simulink model "blast_module_casperize"  (R2019a)
settings: Solver=VariableStepDiscrete  StartTime=0.0  StopTime=10.0  RelTol=1e-3
undefined symbols (not defined in the file): I, pfb_coeff_gen_calc, Q
libraries: xbsIndex_r4 x5938, casper_library_misc x46, casper_library_delays x20, xrbsSSR_Library x9, xps_library x2, casper_library_reorder x2
(part 1 of 83)
settings Model: Creator=root  LastModifiedBy=jackh
settings DataIOCC: LimitDataPoints=on  SaveFormat=Array  ReturnWorkspaceOutputs=off
settings OptimizationCC: DefaultParameterBehavior=Inlined  ExpressionDepthLimit=2147483647  LifeSpan=inf
settings DebuggingCC: UnderspecifiedInitializationDetection=Classic  MergeDetectMultiDrivingBlocksExec=none  SolverPrmCheckMsg=warning  StateNameClashWarn=warning  PregeneratedLibrarySubsystemCodeDiagnostic=none  SFUnexpectedBacktrackingDiag=warning  SFNoUnconditionalDefaultTransitionDiag=warning  SFExecutionAtInitializationDiag=none  ArithmeticOperatorsInVariantConditions=warning
settings HardwareCC: ProdBitPerPointer=32  ProdBitPerSizeT=32  ProdBitPerPtrDiffT=32  ProdLargestAtomicFloat=None  ProdIntDivRoundTo=Undefined  ProdEndianess=Unspecified  ProdWordSize=32  ProdHWDeviceType=32-bit Generic
settings ModelReferenceCC: PropagateSignalLabelsOutOfModel=off
settings SFSimCC: SimUseLocalCustomCode=off
settings RTWCC: RTWUseLocalCustomCode=off
settings CodeAppCC: StateflowObjectComments=on
settings GRTTargetCC: TargetLangStandard=C89/C90 (ANSI)  GeneratePreprocessorConditionals=Disable all
settings ConfigComp: CovMetricSettings=dw  CovHtmlReporting=on  CovSaveCumulativeToWorkspaceVar=on  CovSaveSingleToWorkspaceVar=on  CovExternalEMLEnable=off

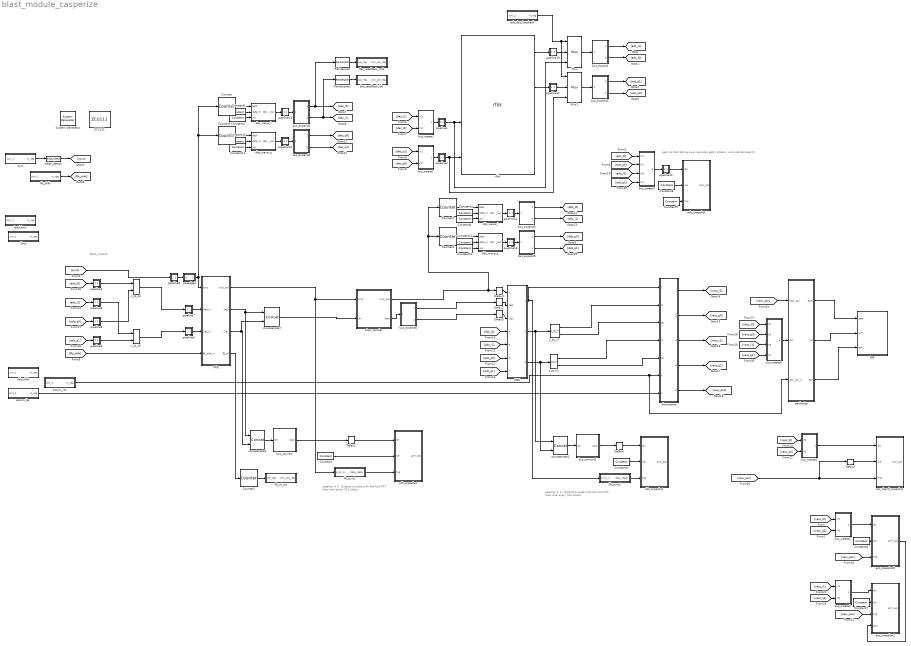
== system blast_module_casperize ==
  note: pack so that taking even samples gets I stream, and odd samples Q
  note: blast_module
  note: Latency = 2. Outputs a pulse with the first FFT,
      | then one every 512 clocks
  note: Latency = 2. Outputs a pulse with the first FFT,
      | then one every 512 clocks
  " System Generator" : xbsIndex_r4/ System Generator  Tag=genX  xilinxfamily=zynquplusRFSOC  part=xczu28dr  speed=-2-e  package=ffvg1517  synthesis_tool=XST  clock_wrapper=Clock Enables  directory=/home/jackh/src/umanc/souk/blast_module_casperize/sysgen  proj_type=Vivado  Synth_file=Vivado Synthesis Defaults  Impl_file=Vivado Implementation Defaults  testbench=off  simulink_period=1  sysclk_period=4.069  dcm_input_clock_period=10  incr_netlist=off  trim_vbits=Everywhere in SubSystem  dbl_ovrd=According to Block Masks  core_generation=According to Block Masks  run_coregen=off  deprecated_control=off  eval_field=0  block_type=sysgen
  Constant{,5..9} (6 alike) : xbsIndex_r4/Constant  const=1.0  gui_display_data_type=Boolean  arith_type=Boolean  n_bits=16  bin_pt=14  preci_type=Single  exp_width=8  frac_width=24  explicit_period=on  period=1  equ=P=C  opselect=C  inp2=PCIN>>17  opr=+  inp1=P  carry=CIN  dbl_ovrd=off  block_type=constant
  Constant{1,3,10,12} (4 alike) : xbsIndex_r4/Constant  const=0  gui_display_data_type=Fixed-point  arith_type=Unsigned  n_bits=32  bin_pt=0  preci_type=Single  exp_width=8  frac_width=24  explicit_period=on  period=1  equ=P=C  opselect=C  inp2=PCIN>>17  opr=+  inp1=P  carry=CIN  dbl_ovrd=off  block_type=constant
  Constant{2,4,11,13} (4 alike) : xbsIndex_r4/Constant  const=0  gui_display_data_type=Boolean  arith_type=Boolean  n_bits=64  bin_pt=0  preci_type=Single  exp_width=8  frac_width=24  explicit_period=on  period=1  equ=P=C  opselect=C  inp2=PCIN>>17  opr=+  inp1=P  carry=CIN  dbl_ovrd=off  block_type=constant
  Counter{,1,3..4} (4 alike) : xbsIndex_r4/Counter  cnt_type=Free Running  cnt_to=Inf  operation=Up  start_count=0  cnt_by_val=1  arith_type=Unsigned  n_bits=17  bin_pt=0  load_pin=off  rst=on  en=off  explicit_period=on  period=1  use_behavioral_HDL=off  implementation=Fabric  dbl_ovrd=off  block_type=counter
  Counter2 : xbsIndex_r4/Counter  cnt_type=Free Running  cnt_to=Inf  operation=Up  start_count=0  cnt_by_val=1  arith_type=Unsigned  n_bits=32  bin_pt=0  load_pin=off  rst=off  en=on  explicit_period=on  period=1  use_behavioral_HDL=off  implementation=Fabric  dbl_ovrd=off  block_type=counter
  DDC : Subsystem
  Delay{1..5} (5 alike) : xbsIndex_r4/Delay  rst=off  infoeditControl=Selection of Reset will increase slice count due to use of real FFs and instead of SRLs  en=off  latency=2  reg_retiming=off  dbl_ovrd=off  block_type=delay
      settings: SourceProductName=Attempt to write the readonly database /home/ugrad/.matlab/R2018a/slblocks_master.db. (attempt to write a readonly database)  xl_area=[18 36 0 0 0 0 0]
  Delay9 : xbsIndex_r4/Delay  rst=off  infoeditControl=Selection of Reset will increase slice count due to use of real FFs and instead of SRLs  en=off  latency=1  reg_retiming=off  dbl_ovrd=off  block_type=delay
      settings: SourceProductName=Attempt to write the readonly database /home/ugrad/.matlab/R2018a/slblocks_master.db. (attempt to write a readonly database)  xl_area=[18 36 0 0 0 0 0]
  Mux : xbsIndex_r4/Mux  inputs=2  en=off  latency=1  precision=Full  arith_type=Unsigned  n_bits=16  bin_pt=14  quantization=Truncate  overflow=Wrap  dbl_ovrd=off  block_type=mux
  Mux1 : xbsIndex_r4/Mux  inputs=2  en=off  latency=1  precision=Full  arith_type=Unsigned  n_bits=16  bin_pt=14  quantization=Truncate  overflow=Wrap  dbl_ovrd=off  block_type=mux
  PFB : Subsystem
  Reinterpret : xbsIndex_r4/Reinterpret  force_arith_type=on  arith_type=Unsigned  force_bin_pt=on  bin_pt=0  block_type=reinterpret
  Reinterpret1 : xbsIndex_r4/Reinterpret  force_arith_type=on  arith_type=Unsigned  force_bin_pt=on  bin_pt=0  block_type=reinterpret
  ZCU111 : xps_library/Platforms/ZCU111  Tag=xps:xsg  hw_sys=ZCU111:xczu28dr  clk_src=adc_clk  clk_rate=245.76  pl_clk_rate=122.88  sample_period=1  synthesis_tool=XST
      settings: SourceProductName=CASPER XPS Blockset
  acc_chan0_snapshot : Subsystem  Tag=casper:snapshot  AncestorBlock=casper_library_scopes/snapshot  mask(snapshot){storage=bram, dram_dimm=2, dram_clock=250, nsamples=13, data_width=64, offset=off, circap=off, value=off, ext_arm=off, ext_circ=off, provide_outputs=on, use_dsp48=off}
      mask prompts: storage "Storage medium"; dram_dimm "DRAM dimm"; dram_clock "DRAM clock rate"; nsamples "Number of Samples (2^?)"; data_width "Data width"; offset "Start delay support"; circap "Circular capture support"; value "Extra value capture support"; ext_arm "External arm support"; ext_circ "External circular capture support"; provide_outputs "Provide outputs"; use_dsp48 "Use DSP48s to implement counters"
      mask help:
      | Standard snap block, but with the following optional extras;
      |  1) Optionally delay the fabric trigger by a user-specified number of valids.
      |  2) Capture continuously after a trigger until a stop pulse is received. Data is captured into BRAM continuously, with old data being overwritten until a stop command is received. Then stop capturing when memory is filled. This enables you to get some data before and some data after the stop pulse. Use the 'tr_en_cnt' register to determine where you are in your vector. 'Addr' register's MSb now indicates 'busy capturing'.
      |  3) Optionally capture a value on an input port to a register at the same time as the first data sample.
      |  4) Implement counters using DSP48Es to save resources.
      mask init:
      | snapshot_init(gcb, ...
      |     'storage', storage, ...
      |     'dram_dimm', dram_dimm, ...
      |     'dram_clock', dram_clock, ...
      |     'nsamples', nsamples, ...
      |     'data_width', data_width, ...
      |     'offset', offset, ...
      |     'circap', circap, ...
      |     'value', value, ...
      |     'ext_arm', ext_arm, ...
      |     'ext_circ', ext_circ, ...
      |     'provide_outputs', 'off', ...
      |     'use_dsp48', use_dsp48);
      settings: AttributesFormatString=|
      | 64 wide, 8192 deep
      | debugID: 9255584
      mask TypeOptions storage: bram | dram
      mask Callback storage: snapshot_callback();
      mask TypeOptions dram_dimm: 1 | 2 | 3 | 4
      mask TypeOptions dram_clock: 200 | 250 | 266 | 300 | 333
      mask TypeOptions data_width: 8 | 16 | 32 | 64 | 128
  acc_snapshot0 : Subsystem  Tag=casper:snapshot  AncestorBlock=casper_library_scopes/snapshot  mask(snapshot){storage=bram, dram_dimm=2, dram_clock=250, nsamples=10, data_width=64, offset=off, circap=off, value=off, ext_arm=off, ext_circ=off, provide_outputs=on, use_dsp48=off}
      mask prompts: storage "Storage medium"; dram_dimm "DRAM dimm"; dram_clock "DRAM clock rate"; nsamples "Number of Samples (2^?)"; data_width "Data width"; offset "Start delay support"; circap "Circular capture support"; value "Extra value capture support"; ext_arm "External arm support"; ext_circ "External circular capture support"; provide_outputs "Provide outputs"; use_dsp48 "Use DSP48s to implement counters"
      mask help:
      | Standard snap block, but with the following optional extras;
      |  1) Optionally delay the fabric trigger by a user-specified number of valids.
      |  2) Capture continuously after a trigger until a stop pulse is received. Data is captured into BRAM continuously, with old data being overwritten until a stop command is received. Then stop capturing when memory is filled. This enables you to get some data before and some data after the stop pulse. Use the 'tr_en_cnt' register to determine where you are in your vector. 'Addr' register's MSb now indicates 'busy capturing'.
      |  3) Optionally capture a value on an input port to a register at the same time as the first data sample.
      |  4) Implement counters using DSP48Es to save resources.
      mask init: same as blast_module_casperize/acc_chan0_snapshot
      settings: AttributesFormatString=|
      | 64 wide, 1024 deep
      | debugID: 50070968
      mask TypeOptions storage: bram | dram
      mask Callback storage: snapshot_callback();
      mask TypeOptions dram_dimm: 1 | 2 | 3 | 4
      mask TypeOptions dram_clock: 200 | 250 | 266 | 300 | 333
      mask TypeOptions data_width: 8 | 16 | 32 | 64 | 128
  acc_snapshot1 : Subsystem  Tag=casper:snapshot  AncestorBlock=casper_library_scopes/snapshot  mask(snapshot){storage=bram, dram_dimm=2, dram_clock=250, nsamples=10, data_width=64, offset=off, circap=off, value=off, ext_arm=on, ext_circ=off, provide_outputs=on, use_dsp48=off}
      mask prompts: storage "Storage medium"; dram_dimm "DRAM dimm"; dram_clock "DRAM clock rate"; nsamples "Number of Samples (2^?)"; data_width "Data width"; offset "Start delay support"; circap "Circular capture support"; value "Extra value capture support"; ext_arm "External arm support"; ext_circ "External circular capture support"; provide_outputs "Provide outputs"; use_dsp48 "Use DSP48s to implement counters"
      mask help:
      | Standard snap block, but with the following optional extras;
      |  1) Optionally delay the fabric trigger by a user-specified number of valids.
      |  2) Capture continuously after a trigger until a stop pulse is received. Data is captured into BRAM continuously, with old data being overwritten until a stop command is received. Then stop capturing when memory is filled. This enables you to get some data before and some data after the stop pulse. Use the 'tr_en_cnt' register to determine where you are in your vector. 'Addr' register's MSb now indicates 'busy capturing'.
      |  3) Optionally capture a value on an input port to a register at the same time as the first data sample.
      |  4) Implement counters using DSP48Es to save resources.
      mask init: same as blast_module_casperize/acc_chan0_snapshot
      settings: AttributesFormatString=|
      | 64 wide, 1024 deep
      | debugID: 50070969
      mask TypeOptions storage: bram | dram
      mask Callback storage: snapshot_callback();
      mask TypeOptions dram_dimm: 1 | 2 | 3 | 4
      mask TypeOptions dram_clock: 200 | 250 | 266 | 300 | 333
      mask TypeOptions data_width: 8 | 16 | 32 | 64 | 128
  accum_len : Subsystem  Tag=xps:sw_reg  AncestorBlock=xps_library/Memory/software_register  mask(swreg){io_dir=From Processor, io_delay=0, init_val=0, sample_period=1, names=reg, bitwidths=24, bin_pts=0, arith_types=0, sim_port=on, show_format=on}
      mask prompts: io_dir "I/O direction"; io_delay "I/O delay"; init_val "Initial Value"; sample_period "Sample period"; names "Bitfield names [msb...lsb]"; bitwidths "Bitfield widths"; bin_pts "Bitfield binary pts"; arith_types "Bitfield types, ufix=0, fix=1, bool=2"; sim_port "Provide sim input/output?"; show_format "Print format string?"
      mask help: A 32-bit software-accessible register. Can be divided into bitfields of varying widths and types using the fields in the block mask.
      mask init:
      | swreg_init(gcb)
      settings: AttributesFormatString=1input:uf24.0 = 24 bits
      mask TypeOptions io_dir: To Processor | From Processor
      mask Callback io_dir:
      | mask_enables = get_param(gcb, 'MaskEnables');
      | mask_names = get_param(gcb, 'MaskNames');
      | if strcmp(get_param(gcb, 'io_dir'), 'To Processor'),
      |     mask_enables{ismember(mask_names, 'sample_period')} = 'off';
      | else
      |     mask_enables{ismember(mask_names, 'sample_period')} = 'on';
      | end
      | set_param(gcb, 'MaskEnables', mask_enables);
      mask DialogControl ParameterTabVar0 Prompt: Setup
  accum_rst : Subsystem  Tag=xps:sw_reg  AncestorBlock=xps_library/Memory/software_register  mask(swreg){io_dir=From Processor, io_delay=0, init_val=0, sample_period=1, names=reg, bitwidths=1, bin_pts=0, arith_types=2, sim_port=on, show_format=on}
      mask prompts: io_dir "I/O direction"; io_delay "I/O delay"; init_val "Initial Value"; sample_period "Sample period"; names "Bitfield names [msb...lsb]"; bitwidths "Bitfield widths"; bin_pts "Bitfield binary pts"; arith_types "Bitfield types, ufix=0, fix=1, bool=2"; sim_port "Provide sim input/output?"; show_format "Print format string?"
      mask help: A 32-bit software-accessible register. Can be divided into bitfields of varying widths and types using the fields in the block mask.
      mask init:
      | swreg_init(gcb)
      settings: AttributesFormatString=1input:b = 1 bits
      mask TypeOptions io_dir: To Processor | From Processor
      mask Callback io_dir:
      | mask_enables = get_param(gcb, 'MaskEnables');
      | mask_names = get_param(gcb, 'MaskNames');
      | if strcmp(get_param(gcb, 'io_dir'), 'To Processor'),
      |     mask_enables{ismember(mask_names, 'sample_period')} = 'off';
      | else
      |     mask_enables{ismember(mask_names, 'sample_period')} = 'on';
      | end
      | set_param(gcb, 'MaskEnables', mask_enables);
      mask DialogControl ParameterTabVar0 Prompt: Setup
  adc_dac_loopback : Subsystem  Tag=xps:sw_reg  AncestorBlock=xps_library/Memory/software_register  mask(swreg){io_dir=From Processor, io_delay=0, init_val=0, sample_period=1, names=reg, bitwidths=1, bin_pts=0, arith_types=0, sim_port=on, show_format=on}
      mask prompts: io_dir "I/O direction"; io_delay "I/O delay"; init_val "Initial Value"; sample_period "Sample period"; names "Bitfield names [msb...lsb]"; bitwidths "Bitfield widths"; bin_pts "Bitfield binary pts"; arith_types "Bitfield types, ufix=0, fix=1, bool=2"; sim_port "Provide sim input/output?"; show_format "Print format string?"
      mask help: A 32-bit software-accessible register. Can be divided into bitfields of varying widths and types using the fields in the block mask.
      mask init:
      | swreg_init(gcb)
      settings: AttributesFormatString=1input:uf1.0 = 1 bits
      mask TypeOptions io_dir: To Processor | From Processor
      mask Callback io_dir:
      | mask_enables = get_param(gcb, 'MaskEnables');
      | mask_names = get_param(gcb, 'MaskNames');
      | if strcmp(get_param(gcb, 'io_dir'), 'To Processor'),
      |     mask_enables{ismember(mask_names, 'sample_period')} = 'off';
      | else
      |     mask_enables{ismember(mask_names, 'sample_period')} = 'on';
      | end
      | set_param(gcb, 'MaskEnables', mask_enables);
      mask DialogControl ParameterTabVar0 Prompt: Setup
  adc_snapshot : Subsystem  Tag=casper:snapshot  AncestorBlock=casper_library_scopes/snapshot  mask(snapshot){storage=bram, dram_dimm=2, dram_clock=250, nsamples=11, data_width=64, offset=off, circap=off, value=off, ext_arm=off, ext_circ=off, provide_outputs=on, use_dsp48=off}
      mask prompts: storage "Storage medium"; dram_dimm "DRAM dimm"; dram_clock "DRAM clock rate"; nsamples "Number of Samples (2^?)"; data_width "Data width"; offset "Start delay support"; circap "Circular capture support"; value "Extra value capture support"; ext_arm "External arm support"; ext_circ "External circular capture support"; provide_outputs "Provide outputs"; use_dsp48 "Use DSP48s to implement counters"
      mask help:
      | Standard snap block, but with the following optional extras;
      |  1) Optionally delay the fabric trigger by a user-specified number of valids.
      |  2) Capture continuously after a trigger until a stop pulse is received. Data is captured into BRAM continuously, with old data being overwritten until a stop command is received. Then stop capturing when memory is filled. This enables you to get some data before and some data after the stop pulse. Use the 'tr_en_cnt' register to determine where you are in your vector. 'Addr' register's MSb now indicates 'busy capturing'.
      |  3) Optionally capture a value on an input port to a register at the same time as the first data sample.
      |  4) Implement counters using DSP48Es to save resources.
      mask init: same as blast_module_casperize/acc_chan0_snapshot
      settings: AttributesFormatString=|
      | 64 wide, 2048 deep
      | debugID: 118348857
      mask TypeOptions storage: bram | dram
      mask Callback storage: snapshot_callback();
      mask TypeOptions dram_dimm: 1 | 2 | 3 | 4
      mask TypeOptions dram_clock: 200 | 250 | 266 | 300 | 333
      mask TypeOptions data_width: 8 | 16 | 32 | 64 | 128
  bins : Subsystem  Tag=xps:sw_reg  AncestorBlock=xps_library/Memory/software_register  mask(swreg){io_dir=From Processor, io_delay=0, init_val=0, sample_period=1, names=reg, bitwidths=10, bin_pts=0, arith_types=0, sim_port=on, show_format=on}
      mask prompts: io_dir "I/O direction"; io_delay "I/O delay"; init_val "Initial Value"; sample_period "Sample period"; names "Bitfield names [msb...lsb]"; bitwidths "Bitfield widths"; bin_pts "Bitfield binary pts"; arith_types "Bitfield types, ufix=0, fix=1, bool=2"; sim_port "Provide sim input/output?"; show_format "Print format string?"
      mask help: A 32-bit software-accessible register. Can be divided into bitfields of varying widths and types using the fields in the block mask.
      mask init:
      | swreg_init(gcb)
      settings: AttributesFormatString=1input:uf10.0 = 10 bits
      mask TypeOptions io_dir: To Processor | From Processor
      mask Callback io_dir:
      | mask_enables = get_param(gcb, 'MaskEnables');
      | mask_names = get_param(gcb, 'MaskNames');
      | if strcmp(get_param(gcb, 'io_dir'), 'To Processor'),
      |     mask_enables{ismember(mask_names, 'sample_period')} = 'off';
      | else
      |     mask_enables{ismember(mask_names, 'sample_period')} = 'on';
      | end
      | set_param(gcb, 'MaskEnables', mask_enables);
      mask DialogControl ParameterTabVar0 Prompt: Setup
  bus_convert : Subsystem  AncestorBlock=casper_library_bus/bus_convert  mask(bus_convert){n_bits_in=[18 18 18 18], bin_pt_in=[17 17 17 17], cmplx=off, n_bits_out=16, bin_pt_out=15, quantization=0, overflow=0, csp_latency=0, of=off, misc=off}
      mask prompts: n_bits_in "input bit widths"; bin_pt_in "input binary points"; cmplx "input complex"; n_bits_out "output bit widths"; bin_pt_out "output binary points"; quantization "quantization strategy (Truncate=0, Round  (unbiased: +/- Inf)=1, Round (unbiased: Even Values)=2)"; overflow "overflow strategy (Wrap=0, Saturate=1, Flag as error=2)"; csp_latency "latency"; of "overflow indication"; misc "misc support"
      mask help: Convert components of busses
      mask init:
      | bus_convert_init(gcb, ...
      |     'n_bits_in', n_bits_in, ...
      |     'bin_pt_in', bin_pt_in, ...
      |     'cmplx', cmplx, ...
      |     'n_bits_out', n_bits_out, ...
      |     'bin_pt_out', bin_pt_out, ...
      |     'quantization', quantization, ...
      |     'overflow', overflow, ...
      |     'csp_latency', csp_latency, ...
      |     'misc', misc, ...
      |     'of', of);
  bus_convert1 : Subsystem  AncestorBlock=casper_library_bus/bus_convert  mask(bus_convert){n_bits_in=[19 19 19 19], bin_pt_in=[18 18 18 18], cmplx=off, n_bits_out=16, bin_pt_out=15, quantization=0, overflow=0, csp_latency=0, of=off, misc=off}
      mask prompts: n_bits_in "input bit widths"; bin_pt_in "input binary points"; cmplx "input complex"; n_bits_out "output bit widths"; bin_pt_out "output binary points"; quantization "quantization strategy (Truncate=0, Round  (unbiased: +/- Inf)=1, Round (unbiased: Even Values)=2)"; overflow "overflow strategy (Wrap=0, Saturate=1, Flag as error=2)"; csp_latency "latency"; of "overflow indication"; misc "misc support"
      mask help: Convert components of busses
      mask init: same as blast_module_casperize/bus_convert
  bus_create : Subsystem  AncestorBlock=casper_library_flow_control/bus_create  mask(bus_create){inputNum=2}
      mask prompts: inputNum "Number of inputs:"
      mask init:
      | bus_create_init(gcb,...
      |     'inputNum', inputNum);
  bus_create1 : Subsystem  AncestorBlock=casper_library_flow_control/bus_create  mask(bus_create){inputNum=2}
      mask prompts: inputNum "Number of inputs:"
      mask init:
      | bus_create_init(gcb,...
      |     'inputNum', inputNum);
  bus_create2 : Subsystem  AncestorBlock=casper_library_flow_control/bus_create  mask(bus_create){inputNum=2}
      mask prompts: inputNum "Number of inputs:"
      mask init:
      | bus_create_init(gcb,...
      |     'inputNum', inputNum);
  bus_create3 : Subsystem  AncestorBlock=casper_library_flow_control/bus_create  mask(bus_create){inputNum=2}
      mask prompts: inputNum "Number of inputs:"
      mask init:
      | bus_create_init(gcb,...
      |     'inputNum', inputNum);
  bus_create4 : Subsystem  AncestorBlock=casper_library_flow_control/bus_create  mask(bus_create){inputNum=4}
      mask prompts: inputNum "Number of inputs:"
      mask init:
      | bus_create_init(gcb,...
      |     'inputNum', inputNum);
  bus_create5 : Subsystem  AncestorBlock=casper_library_flow_control/bus_create  mask(bus_create){inputNum=2}
      mask prompts: inputNum "Number of inputs:"
      mask init:
      | bus_create_init(gcb,...
      |     'inputNum', inputNum);
  bus_create6 : Subsystem  AncestorBlock=casper_library_flow_control/bus_create  mask(bus_create){inputNum=4}
      mask prompts: inputNum "Number of inputs:"
      mask init:
      | bus_create_init(gcb,...
      |     'inputNum', inputNum);
  bus_expand : Subsystem  AncestorBlock=casper_library_flow_control/bus_expand  mask(bus_expand){mode=divisions of equal size, outputNum=2, outputWidth=16, outputBinaryPt=15, outputArithmeticType=1, show_format=off, outputToWorkspace=off, variablePrefix=out, outputToModelAsWell=on}
      mask prompts: outputNum "Number of outputs:"; outputWidth "Output width:"; outputBinaryPt "Output binary point position:"; outputArithmeticType "Output arithmetic type (ufix=0, fix=1, bool=2):"; show_format "Print format string?"; outputToWorkspace "Output to workspace?"; variablePrefix "Variable name prefix:"; outputToModelAsWell "Output to model as well?"
      mask help:
      | Expands a 'bus' made using a bus_create or Xilinx
      | concat block.
      | The input will be divided into the specified number
      | of outputs with the specified arithmetic types.
      | Divisions are made from most significant bit.
      mask init:
      | bus_expand_init(gcb,...
      |     'mode', mode, ...
      |     'outputNum', outputNum, ...
      |     'outputWidth', outputWidth, ...
      |     'outputBinaryPt', outputBinaryPt, ...
      |     'outputArithmeticType', outputArithmeticType, ...
      |     'show_format', show_format, ...
      |     'outputToWorkspace', outputToWorkspace, ...
      |     'variablePrefix', variablePrefix, ...
      |     'outputToModelAsWell', outputToModelAsWell);
      settings: AttributesFormatString=2 outputs
      mask TypeOptions mode: divisions of equal size | divisions of arbitrary size
      mask Callback mode: bus_expand_callback();
      mask Callback outputWidth: bus_expand_callback();
      mask Callback outputToWorkspace: bus_expand_callback();
  bus_expand1 : Subsystem  AncestorBlock=casper_library_flow_control/bus_expand  mask(bus_expand){mode=divisions of equal size, outputNum=2, outputWidth=16, outputBinaryPt=15, outputArithmeticType=1, show_format=off, outputToWorkspace=off, variablePrefix=out, outputToModelAsWell=on}
      mask prompts: outputNum "Number of outputs:"; outputWidth "Output width:"; outputBinaryPt "Output binary point position:"; outputArithmeticType "Output arithmetic type (ufix=0, fix=1, bool=2):"; show_format "Print format string?"; outputToWorkspace "Output to workspace?"; variablePrefix "Variable name prefix:"; outputToModelAsWell "Output to model as well?"
      mask help:
      | Expands a 'bus' made using a bus_create or Xilinx
      | concat block.
      | The input will be divided into the specified number
      | of outputs with the specified arithmetic types.
      | Divisions are made from most significant bit.
      mask init: same as blast_module_casperize/bus_expand
      settings: AttributesFormatString=2 outputs
      mask TypeOptions mode: divisions of equal size | divisions of arbitrary size
      mask Callback mode: bus_expand_callback();
      mask Callback outputWidth: bus_expand_callback();
      mask Callback outputToWorkspace: bus_expand_callback();
  bus_expand2 : Subsystem  AncestorBlock=casper_library_flow_control/bus_expand  mask(bus_expand){mode=divisions of equal size, outputNum=2, outputWidth=16, outputBinaryPt=15, outputArithmeticType=1, show_format=off, outputToWorkspace=off, variablePrefix=out, outputToModelAsWell=on}
      mask prompts: outputNum "Number of outputs:"; outputWidth "Output width:"; outputBinaryPt "Output binary point position:"; outputArithmeticType "Output arithmetic type (ufix=0, fix=1, bool=2):"; show_format "Print format string?"; outputToWorkspace "Output to workspace?"; variablePrefix "Variable name prefix:"; outputToModelAsWell "Output to model as well?"
      mask help:
      | Expands a 'bus' made using a bus_create or Xilinx
      | concat block.
      | The input will be divided into the specified number
      | of outputs with the specified arithmetic types.
      | Divisions are made from most significant bit.
      mask init: same as blast_module_casperize/bus_expand
      settings: AttributesFormatString=2 outputs
      mask TypeOptions mode: divisions of equal size | divisions of arbitrary size
      mask Callback mode: bus_expand_callback();
      mask Callback outputWidth: bus_expand_callback();
      mask Callback outputToWorkspace: bus_expand_callback();
  bus_expand3 : Subsystem  AncestorBlock=casper_library_flow_control/bus_expand  mask(bus_expand){mode=divisions of equal size, outputNum=2, outputWidth=16, outputBinaryPt=15, outputArithmeticType=1, show_format=off, outputToWorkspace=off, variablePrefix=out, outputToModelAsWell=on}
      mask prompts: outputNum "Number of outputs:"; outputWidth "Output width:"; outputBinaryPt "Output binary point position:"; outputArithmeticType "Output arithmetic type (ufix=0, fix=1, bool=2):"; show_format "Print format string?"; outputToWorkspace "Output to workspace?"; variablePrefix "Variable name prefix:"; outputToModelAsWell "Output to model as well?"
      mask help:
      | Expands a 'bus' made using a bus_create or Xilinx
      | concat block.
      | The input will be divided into the specified number
      | of outputs with the specified arithmetic types.
      | Divisions are made from most significant bit.
      mask init: same as blast_module_casperize/bus_expand
      settings: AttributesFormatString=2 outputs
      mask TypeOptions mode: divisions of equal size | divisions of arbitrary size
      mask Callback mode: bus_expand_callback();
      mask Callback outputWidth: bus_expand_callback();
      mask Callback outputToWorkspace: bus_expand_callback();
  bus_expand4 : Subsystem  AncestorBlock=casper_library_flow_control/bus_expand  mask(bus_expand){mode=divisions of equal size, outputNum=2, outputWidth=16, outputBinaryPt=15, outputArithmeticType=1, show_format=off, outputToWorkspace=off, variablePrefix=out, outputToModelAsWell=on}
      mask prompts: outputNum "Number of outputs:"; outputWidth "Output width:"; outputBinaryPt "Output binary point position:"; outputArithmeticType "Output arithmetic type (ufix=0, fix=1, bool=2):"; show_format "Print format string?"; outputToWorkspace "Output to workspace?"; variablePrefix "Variable name prefix:"; outputToModelAsWell "Output to model as well?"
      mask help:
      | Expands a 'bus' made using a bus_create or Xilinx
      | concat block.
      | The input will be divided into the specified number
      | of outputs with the specified arithmetic types.
      | Divisions are made from most significant bit.
      mask init: same as blast_module_casperize/bus_expand
      settings: AttributesFormatString=2 outputs
      mask TypeOptions mode: divisions of equal size | divisions of arbitrary size
      mask Callback mode: bus_expand_callback();
      mask Callback outputWidth: bus_expand_callback();
      mask Callback outputToWorkspace: bus_expand_callback();
  bus_expand5 : Subsystem  AncestorBlock=casper_library_flow_control/bus_expand  mask(bus_expand){mode=divisions of equal size, outputNum=2, outputWidth=16, outputBinaryPt=15, outputArithmeticType=1, show_format=off, outputToWorkspace=off, variablePrefix=out, outputToModelAsWell=on}
      mask prompts: outputNum "Number of outputs:"; outputWidth "Output width:"; outputBinaryPt "Output binary point position:"; outputArithmeticType "Output arithmetic type (ufix=0, fix=1, bool=2):"; show_format "Print format string?"; outputToWorkspace "Output to workspace?"; variablePrefix "Variable name prefix:"; outputToModelAsWell "Output to model as well?"
      mask help:
      | Expands a 'bus' made using a bus_create or Xilinx
      | concat block.
      | The input will be divided into the specified number
      | of outputs with the specified arithmetic types.
      | Divisions are made from most significant bit.
      mask init: same as blast_module_casperize/bus_expand
      settings: AttributesFormatString=2 outputs
      mask TypeOptions mode: divisions of equal size | divisions of arbitrary size
      mask Callback mode: bus_expand_callback();
      mask Callback outputWidth: bus_expand_callback();
      mask Callback outputToWorkspace: bus_expand_callback();
  bus_expand6 : Subsystem  AncestorBlock=casper_library_flow_control/bus_expand  mask(bus_expand){mode=divisions of equal size, outputNum=2, outputWidth=36, outputBinaryPt=0, outputArithmeticType=0, show_format=off, outputToWorkspace=off, variablePrefix=out, outputToModelAsWell=on}
      mask prompts: outputNum "Number of outputs:"; outputWidth "Output width:"; outputBinaryPt "Output binary point position:"; outputArithmeticType "Output arithmetic type (ufix=0, fix=1, bool=2):"; show_format "Print format string?"; outputToWorkspace "Output to workspace?"; variablePrefix "Variable name prefix:"; outputToModelAsWell "Output to model as well?"
      mask help:
      | Expands a 'bus' made using a bus_create or Xilinx
      | concat block.
      | The input will be divided into the specified number
      | of outputs with the specified arithmetic types.
      | Divisions are made from most significant bit.
      mask init: same as blast_module_casperize/bus_expand
      settings: AttributesFormatString=2 outputs
      mask TypeOptions mode: divisions of equal size | divisions of arbitrary size
      mask Callback mode: bus_expand_callback();
      mask Callback outputWidth: bus_expand_callback();
      mask Callback outputToWorkspace: bus_expand_callback();
  c_to_ri1 : casper_library_misc/c_to_ri  n_bits=19  bin_pt=17
      settings: AttributesFormatString=19_17 r/i  SourceProductName=CASPER DSP Blockset
  c_to_ri7 : casper_library_misc/c_to_ri  n_bits=19  bin_pt=17
      settings: AttributesFormatString=19_17 r/i  SourceProductName=CASPER DSP Blockset
  chan_reorder : Subsystem
  concatenate1 : xbsIndex_r4/Concat  num_inputs=2  dbl_ovrd=off  block_type=concat
      settings: SourceProductName=Attempt to write the readonly database /home/ugrad/.matlab/R2018a/slblocks_master.db. (attempt to write a readonly database)
  concatenate2 : xbsIndex_r4/Concat  num_inputs=2  dbl_ovrd=off  block_type=concat
      settings: SourceProductName=Attempt to write the readonly database /home/ugrad/.matlab/R2018a/slblocks_master.db. (attempt to write a readonly database)
  concatenate7 : xbsIndex_r4/Concat  num_inputs=2  dbl_ovrd=off  block_type=concat
      settings: SourceProductName=Attempt to write the readonly database /home/ugrad/.matlab/R2018a/slblocks_master.db. (attempt to write a readonly database)
  dac_readback_lsb : Subsystem  Tag=xps:sw_reg  AncestorBlock=xps_library/Memory/software_register  mask(swreg){io_dir=To Processor, io_delay=0, init_val=0, sample_period=1, names=reg, bitwidths=16, bin_pts=0, arith_types=0, sim_port=on, show_format=on}
      mask prompts: io_dir "I/O direction"; io_delay "I/O delay"; init_val "Initial Value"; sample_period "Sample period"; names "Bitfield names [msb...lsb]"; bitwidths "Bitfield widths"; bin_pts "Bitfield binary pts"; arith_types "Bitfield types, ufix=0, fix=1, bool=2"; sim_port "Provide sim input/output?"; show_format "Print format string?"
      mask help: A 32-bit software-accessible register. Can be divided into bitfields of varying widths and types using the fields in the block mask.
      mask init:
      | swreg_init(gcb)
      settings: AttributesFormatString=1output:uf16.0 = 16 bits
      mask TypeOptions io_dir: To Processor | From Processor
      mask Callback io_dir:
      | mask_enables = get_param(gcb, 'MaskEnables');
      | mask_names = get_param(gcb, 'MaskNames');
      | if strcmp(get_param(gcb, 'io_dir'), 'To Processor'),
      |     mask_enables{ismember(mask_names, 'sample_period')} = 'off';
      | else
      |     mask_enables{ismember(mask_names, 'sample_period')} = 'on';
      | end
      | set_param(gcb, 'MaskEnables', mask_enables);
      mask DialogControl ParameterTabVar0 Prompt: Setup
  dac_readback_msb : Subsystem  Tag=xps:sw_reg  AncestorBlock=xps_library/Memory/software_register  mask(swreg){io_dir=To Processor, io_delay=0, init_val=0, sample_period=1, names=reg, bitwidths=16, bin_pts=0, arith_types=0, sim_port=on, show_format=on}
      mask prompts: io_dir "I/O direction"; io_delay "I/O delay"; init_val "Initial Value"; sample_period "Sample period"; names "Bitfield names [msb...lsb]"; bitwidths "Bitfield widths"; bin_pts "Bitfield binary pts"; arith_types "Bitfield types, ufix=0, fix=1, bool=2"; sim_port "Provide sim input/output?"; show_format "Print format string?"
      mask help: A 32-bit software-accessible register. Can be divided into bitfields of varying widths and types using the fields in the block mask.
      mask init:
      | swreg_init(gcb)
      settings: AttributesFormatString=1output:uf16.0 = 16 bits
      mask TypeOptions io_dir: To Processor | From Processor
      mask Callback io_dir:
      | mask_enables = get_param(gcb, 'MaskEnables');
      | mask_names = get_param(gcb, 'MaskNames');
      | if strcmp(get_param(gcb, 'io_dir'), 'To Processor'),
      |     mask_enables{ismember(mask_names, 'sample_period')} = 'off';
      | else
      |     mask_enables{ismember(mask_names, 'sample_period')} = 'on';
      | end
      | set_param(gcb, 'MaskEnables', mask_enables);
      mask DialogControl ParameterTabVar0 Prompt: Setup
  dac_wave_i : Subsystem  Tag=xps:bram  AncestorBlock=xps_library/Memory/shared_bram  mask{arith_type=Unsigned, addr_width=17, data_width=32, reg_prim_output=off, reg_core_output=off, optimization=Minimum_Area, data_bin_pt=0, init_vals=[0:2^10-1], sample_rate=1}
      mask prompts: arith_type "Output Data Type"; addr_width "Address width"; data_width "Data Width"; reg_prim_output "Register Primitive Output"; reg_core_output "Register Core Output"; data_bin_pt "Data Binary Point"; init_vals "Initial values (simulation only)"; sample_rate "Sample rate"
      mask init:
      | shared_bram_mask;
      mask TypeOptions arith_type: Unsigned | Signed  (2's comp)
      mask TypeOptions data_width: 8 | 16 | 32 | 64 | 128
      mask TypeOptions optimization: Minimum_Area | Low_Power
  dac_wave_q : Subsystem  Tag=xps:bram  AncestorBlock=xps_library/Memory/shared_bram  mask{arith_type=Unsigned, addr_width=17, data_width=32, reg_prim_output=off, reg_core_output=off, optimization=Minimum_Area, data_bin_pt=0, init_vals=[0:2^10-1], sample_rate=1}
      mask prompts: arith_type "Output Data Type"; addr_width "Address width"; data_width "Data Width"; reg_prim_output "Register Primitive Output"; reg_core_output "Register Core Output"; data_bin_pt "Data Binary Point"; init_vals "Initial values (simulation only)"; sample_rate "Sample rate"
      mask init:
      | shared_bram_mask;
      mask TypeOptions arith_type: Unsigned | Signed  (2's comp)
      mask TypeOptions data_width: 8 | 16 | 32 | 64 | 128
      mask TypeOptions optimization: Minimum_Area | Low_Power
  ddc_snapshot : Subsystem  Tag=casper:snapshot  AncestorBlock=casper_library_scopes/snapshot  mask(snapshot){storage=bram, dram_dimm=2, dram_clock=250, nsamples=12, data_width=64, offset=off, circap=off, value=off, ext_arm=off, ext_circ=off, provide_outputs=on, use_dsp48=off}
      mask prompts: storage "Storage medium"; dram_dimm "DRAM dimm"; dram_clock "DRAM clock rate"; nsamples "Number of Samples (2^?)"; data_width "Data width"; offset "Start delay support"; circap "Circular capture support"; value "Extra value capture support"; ext_arm "External arm support"; ext_circ "External circular capture support"; provide_outputs "Provide outputs"; use_dsp48 "Use DSP48s to implement counters"
      mask help:
      | Standard snap block, but with the following optional extras;
      |  1) Optionally delay the fabric trigger by a user-specified number of valids.
      |  2) Capture continuously after a trigger until a stop pulse is received. Data is captured into BRAM continuously, with old data being overwritten until a stop command is received. Then stop capturing when memory is filled. This enables you to get some data before and some data after the stop pulse. Use the 'tr_en_cnt' register to determine where you are in your vector. 'Addr' register's MSb now indicates 'busy capturing'.
      |  3) Optionally capture a value on an input port to a register at the same time as the first data sample.
      |  4) Implement counters using DSP48Es to save resources.
      mask init: same as blast_module_casperize/acc_chan0_snapshot
      settings: AttributesFormatString=|
      | 64 wide, 4096 deep
      | debugID: 95009402
      mask TypeOptions storage: bram | dram
      mask Callback storage: snapshot_callback();
      mask TypeOptions dram_dimm: 1 | 2 | 3 | 4
      mask TypeOptions dram_clock: 200 | 250 | 266 | 300 | 333
      mask TypeOptions data_width: 8 | 16 | 32 | 64 | 128
  dds_shift : Subsystem  Tag=xps:sw_reg  AncestorBlock=xps_library/Memory/software_register  mask(swreg){io_dir=From Processor, io_delay=0, init_val=0, sample_period=1, names=reg, bitwidths=9, bin_pts=0, arith_types=0, sim_port=on, show_format=on}
      mask prompts: io_dir "I/O direction"; io_delay "I/O delay"; init_val "Initial Value"; sample_period "Sample period"; names "Bitfield names [msb...lsb]"; bitwidths "Bitfield widths"; bin_pts "Bitfield binary pts"; arith_types "Bitfield types, ufix=0, fix=1, bool=2"; sim_port "Provide sim input/output?"; show_format "Print format string?"
      mask help: A 32-bit software-accessible register. Can be divided into bitfields of varying widths and types using the fields in the block mask.
      mask init:
      | swreg_init(gcb)
      settings: AttributesFormatString=1input:uf9.0 = 9 bits
      mask TypeOptions io_dir: To Processor | From Processor
      mask Callback io_dir:
      | mask_enables = get_param(gcb, 'MaskEnables');
      | mask_names = get_param(gcb, 'MaskNames');
      | if strcmp(get_param(gcb, 'io_dir'), 'To Processor'),
      |     mask_enables{ismember(mask_names, 'sample_period')} = 'off';
      | else
      |     mask_enables{ismember(mask_names, 'sample_period')} = 'on';
      | end
      | set_param(gcb, 'MaskEnables', mask_enables);
      mask DialogControl ParameterTabVar0 Prompt: Setup
  dds_wave_i : Subsystem  Tag=xps:bram  AncestorBlock=xps_library/Memory/shared_bram  mask{arith_type=Unsigned, addr_width=17, data_width=32, reg_prim_output=off, reg_core_output=off, optimization=Minimum_Area, data_bin_pt=0, init_vals=[0:2^10-1], sample_rate=1}
      mask prompts: arith_type "Output Data Type"; addr_width "Address width"; data_width "Data Width"; reg_prim_output "Register Primitive Output"; reg_core_output "Register Core Output"; data_bin_pt "Data Binary Point"; init_vals "Initial values (simulation only)"; sample_rate "Sample rate"
      mask init:
      | shared_bram_mask;
      mask TypeOptions arith_type: Unsigned | Signed  (2's comp)
      mask TypeOptions data_width: 8 | 16 | 32 | 64 | 128
      mask TypeOptions optimization: Minimum_Area | Low_Power
  dds_wave_q : Subsystem  Tag=xps:bram  AncestorBlock=xps_library/Memory/shared_bram  mask{arith_type=Unsigned, addr_width=17, data_width=32, reg_prim_output=off, reg_core_output=off, optimization=Minimum_Area, data_bin_pt=0, init_vals=[0:2^10-1], sample_rate=1}
      mask prompts: arith_type "Output Data Type"; addr_width "Address width"; data_width "Data Width"; reg_prim_output "Register Primitive Output"; reg_core_output "Register Core Output"; data_bin_pt "Data Binary Point"; init_vals "Initial values (simulation only)"; sample_rate "Sample rate"
      mask init:
      | shared_bram_mask;
      mask TypeOptions arith_type: Unsigned | Signed  (2's comp)
      mask TypeOptions data_width: 8 | 16 | 32 | 64 | 128
      mask TypeOptions optimization: Minimum_Area | Low_Power
  downsamp : Subsystem
  edge_detect : casper_library_misc/edge_detect  edge=Rising  polarity=Active High  x_in=[0 0.08 0.08 0.16 0.16 0.24 0.24 0.32 0.32 0.4]  y_in="[-1 -1  1  1  1  1  1  1  1  1]"  x_out=[0.6 0.68 0.68 0.76 0.76 0.84 0.84 0.92 0.92 1]  y_out="[-1 -1  1  1 -1 -1 -1 -1 -1 -1]"
  fft_of_cnt : Subsystem  Tag=xps:sw_reg  AncestorBlock=xps_library/Memory/software_register  mask(swreg){io_dir=To Processor, io_delay=0, init_val=0, sample_period=1, names=reg, bitwidths=32, bin_pts=0, arith_types=0, sim_port=on, show_format=on}
      mask prompts: io_dir "I/O direction"; io_delay "I/O delay"; init_val "Initial Value"; sample_period "Sample period"; names "Bitfield names [msb...lsb]"; bitwidths "Bitfield widths"; bin_pts "Bitfield binary pts"; arith_types "Bitfield types, ufix=0, fix=1, bool=2"; sim_port "Provide sim input/output?"; show_format "Print format string?"
      mask help: A 32-bit software-accessible register. Can be divided into bitfields of varying widths and types using the fields in the block mask.
      mask init:
      | swreg_init(gcb)
      settings: AttributesFormatString=1output:uf32.0 = 32 bits
      mask TypeOptions io_dir: To Processor | From Processor
      mask Callback io_dir:
      | mask_enables = get_param(gcb, 'MaskEnables');
      | mask_names = get_param(gcb, 'MaskNames');
      | if strcmp(get_param(gcb, 'io_dir'), 'To Processor'),
      |     mask_enables{ismember(mask_names, 'sample_period')} = 'off';
      | else
      |     mask_enables{ismember(mask_names, 'sample_period')} = 'on';
      | end
      | set_param(gcb, 'MaskEnables', mask_enables);
      mask DialogControl ParameterTabVar0 Prompt: Setup
  fft_shift : Subsystem  Tag=xps:sw_reg  AncestorBlock=xps_library/Memory/software_register  mask(swreg){io_dir=From Processor, io_delay=0, init_val=0, sample_period=1, names=reg, bitwidths=10, bin_pts=0, arith_types=0, sim_port=on, show_format=on}
      mask prompts: io_dir "I/O direction"; io_delay "I/O delay"; init_val "Initial Value"; sample_period "Sample period"; names "Bitfield names [msb...lsb]"; bitwidths "Bitfield widths"; bin_pts "Bitfield binary pts"; arith_types "Bitfield types, ufix=0, fix=1, bool=2"; sim_port "Provide sim input/output?"; show_format "Print format string?"
      mask help: A 32-bit software-accessible register. Can be divided into bitfields of varying widths and types using the fields in the block mask.
      mask init:
      | swreg_init(gcb)
      settings: AttributesFormatString=1input:uf10.0 = 10 bits
      mask TypeOptions io_dir: To Processor | From Processor
      mask Callback io_dir:
      | mask_enables = get_param(gcb, 'MaskEnables');
      | mask_names = get_param(gcb, 'MaskNames');
      | if strcmp(get_param(gcb, 'io_dir'), 'To Processor'),
      |     mask_enables{ismember(mask_names, 'sample_period')} = 'off';
      | else
      |     mask_enables{ismember(mask_names, 'sample_period')} = 'on';
      | end
      | set_param(gcb, 'MaskEnables', mask_enables);
      mask DialogControl ParameterTabVar0 Prompt: Setup
  fft_sync1 : Subsystem
  fft_sync2 : Subsystem
  load_bins : Subsystem  Tag=xps:sw_reg  AncestorBlock=xps_library/Memory/software_register  mask(swreg){io_dir=From Processor, io_delay=0, init_val=0, sample_period=1, names=reg, bitwidths=11, bin_pts=0, arith_types=0, sim_port=on, show_format=on}
      mask prompts: io_dir "I/O direction"; io_delay "I/O delay"; init_val "Initial Value"; sample_period "Sample period"; names "Bitfield names [msb...lsb]"; bitwidths "Bitfield widths"; bin_pts "Bitfield binary pts"; arith_types "Bitfield types, ufix=0, fix=1, bool=2"; sim_port "Provide sim input/output?"; show_format "Print format string?"
      mask help: A 32-bit software-accessible register. Can be divided into bitfields of varying widths and types using the fields in the block mask.
      mask init:
      | swreg_init(gcb)
      settings: AttributesFormatString=1input:uf11.0 = 11 bits
      mask TypeOptions io_dir: To Processor | From Processor
      mask Callback io_dir:
      | mask_enables = get_param(gcb, 'MaskEnables');
      | mask_names = get_param(gcb, 'MaskNames');
      | if strcmp(get_param(gcb, 'io_dir'), 'To Processor'),
      |     mask_enables{ismember(mask_names, 'sample_period')} = 'off';
      | else
      |     mask_enables{ismember(mask_names, 'sample_period')} = 'on';
      | end
      | set_param(gcb, 'MaskEnables', mask_enables);
      mask DialogControl ParameterTabVar0 Prompt: Setup
  packetize : Subsystem
  pfb_snapshot : Subsystem  Tag=casper:snapshot  AncestorBlock=casper_library_scopes/snapshot  mask(snapshot){storage=bram, dram_dimm=2, dram_clock=250, nsamples=12, data_width=64, offset=off, circap=off, value=off, ext_arm=off, ext_circ=off, provide_outputs=on, use_dsp48=off}
      mask prompts: storage "Storage medium"; dram_dimm "DRAM dimm"; dram_clock "DRAM clock rate"; nsamples "Number of Samples (2^?)"; data_width "Data width"; offset "Start delay support"; circap "Circular capture support"; value "Extra value capture support"; ext_arm "External arm support"; ext_circ "External circular capture support"; provide_outputs "Provide outputs"; use_dsp48 "Use DSP48s to implement counters"
      mask help:
      | Standard snap block, but with the following optional extras;
      |  1) Optionally delay the fabric trigger by a user-specified number of valids.
      |  2) Capture continuously after a trigger until a stop pulse is received. Data is captured into BRAM continuously, with old data being overwritten until a stop command is received. Then stop capturing when memory is filled. This enables you to get some data before and some data after the stop pulse. Use the 'tr_en_cnt' register to determine where you are in your vector. 'Addr' register's MSb now indicates 'busy capturing'.
      |  3) Optionally capture a value on an input port to a register at the same time as the first data sample.
      |  4) Implement counters using DSP48Es to save resources.
      mask init: same as blast_module_casperize/acc_chan0_snapshot
      settings: AttributesFormatString=|
      | 64 wide, 4096 deep
      | debugID: 95009402
      mask TypeOptions storage: bram | dram
      mask Callback storage: snapshot_callback();
      mask TypeOptions dram_dimm: 1 | 2 | 3 | 4
      mask TypeOptions dram_clock: 200 | 250 | 266 | 300 | 333
      mask TypeOptions data_width: 8 | 16 | 32 | 64 | 128
  pipeline1 : Subsystem  AncestorBlock=casper_library_delays/pipeline  mask(pipeline){csp_latency=1}
      mask prompts: csp_latency "Latency"
      mask help:
      | An explicitly laid-out delay line to avoid mapping to SRL16s
      | for use in pipelining to help achieve timing closure.
      mask init:
      | pipeline_init(gcb,'latency',csp_latency);
      settings: AttributesFormatString=Latency = %<latency>
      mask Display:
      | port_label('input', 1, 'd');
      | port_label('output', 1, 'q');
      | disp(['Z^-', num2str(csp_latency)]);
  pipeline10 : Subsystem  AncestorBlock=casper_library_delays/pipeline  mask(pipeline){csp_latency=1}
      mask prompts: csp_latency "Latency"
      mask help:
      | An explicitly laid-out delay line to avoid mapping to SRL16s
      | for use in pipelining to help achieve timing closure.
      mask init:
      | pipeline_init(gcb,'latency',csp_latency);
      settings: AttributesFormatString=Latency = %<latency>
      mask Display:
      | port_label('input', 1, 'd');
      | port_label('output', 1, 'q');
      | disp(['Z^-', num2str(csp_latency)]);
  pipeline11 : Subsystem  AncestorBlock=casper_library_delays/pipeline  mask(pipeline){csp_latency=1}
      mask prompts: csp_latency "Latency"
      mask help:
      | An explicitly laid-out delay line to avoid mapping to SRL16s
      | for use in pipelining to help achieve timing closure.
      mask init:
      | pipeline_init(gcb,'latency',csp_latency);
      settings: AttributesFormatString=Latency = %<latency>
      mask Display:
      | port_label('input', 1, 'd');
      | port_label('output', 1, 'q');
      | disp(['Z^-', num2str(csp_latency)]);
  pipeline12 : Subsystem  AncestorBlock=casper_library_delays/pipeline  mask(pipeline){csp_latency=1}
      mask prompts: csp_latency "Latency"
      mask help:
      | An explicitly laid-out delay line to avoid mapping to SRL16s
      | for use in pipelining to help achieve timing closure.
      mask init:
      | pipeline_init(gcb,'latency',csp_latency);
      settings: AttributesFormatString=Latency = %<latency>
      mask Display:
      | port_label('input', 1, 'd');
      | port_label('output', 1, 'q');
      | disp(['Z^-', num2str(csp_latency)]);
  pipeline13 : Subsystem  AncestorBlock=casper_library_delays/pipeline  mask(pipeline){csp_latency=1}
      mask prompts: csp_latency "Latency"
      mask help:
      | An explicitly laid-out delay line to avoid mapping to SRL16s
      | for use in pipelining to help achieve timing closure.
      mask init:
      | pipeline_init(gcb,'latency',csp_latency);
      settings: AttributesFormatString=Latency = %<latency>
      mask Display:
      | port_label('input', 1, 'd');
      | port_label('output', 1, 'q');
      | disp(['Z^-', num2str(csp_latency)]);
  pipeline14 : Subsystem  AncestorBlock=casper_library_delays/pipeline  mask(pipeline){csp_latency=1}
      mask prompts: csp_latency "Latency"
      mask help:
      | An explicitly laid-out delay line to avoid mapping to SRL16s
      | for use in pipelining to help achieve timing closure.
      mask init:
      | pipeline_init(gcb,'latency',csp_latency);
      settings: AttributesFormatString=Latency = %<latency>
      mask Display:
      | port_label('input', 1, 'd');
      | port_label('output', 1, 'q');
      | disp(['Z^-', num2str(csp_latency)]);
  pipeline15 : Subsystem  AncestorBlock=casper_library_delays/pipeline  mask(pipeline){csp_latency=1}
      mask prompts: csp_latency "Latency"
      mask help:
      | An explicitly laid-out delay line to avoid mapping to SRL16s
      | for use in pipelining to help achieve timing closure.
      mask init:
      | pipeline_init(gcb,'latency',csp_latency);
      settings: AttributesFormatString=Latency = %<latency>
      mask Display:
      | port_label('input', 1, 'd');
      | port_label('output', 1, 'q');
      | disp(['Z^-', num2str(csp_latency)]);
  pipeline16 : Subsystem  AncestorBlock=casper_library_delays/pipeline  mask(pipeline){csp_latency=1}
      mask prompts: csp_latency "Latency"
      mask help:
      | An explicitly laid-out delay line to avoid mapping to SRL16s
      | for use in pipelining to help achieve timing closure.
      mask init:
      | pipeline_init(gcb,'latency',csp_latency);
      settings: AttributesFormatString=Latency = %<latency>
      mask Display:
      | port_label('input', 1, 'd');
      | port_label('output', 1, 'q');
      | disp(['Z^-', num2str(csp_latency)]);
  pipeline2 : Subsystem  AncestorBlock=casper_library_delays/pipeline  mask(pipeline){csp_latency=1}
      mask prompts: csp_latency "Latency"
      mask help:
      | An explicitly laid-out delay line to avoid mapping to SRL16s
      | for use in pipelining to help achieve timing closure.
      mask init:
      | pipeline_init(gcb,'latency',csp_latency);
      settings: AttributesFormatString=Latency = %<latency>
      mask Display:
      | port_label('input', 1, 'd');
      | port_label('output', 1, 'q');
      | disp(['Z^-', num2str(csp_latency)]);
  pipeline3 : Subsystem  AncestorBlock=casper_library_delays/pipeline  mask(pipeline){csp_latency=1}
      mask prompts: csp_latency "Latency"
      mask help:
      | An explicitly laid-out delay line to avoid mapping to SRL16s
      | for use in pipelining to help achieve timing closure.
      mask init:
      | pipeline_init(gcb,'latency',csp_latency);
      settings: AttributesFormatString=Latency = %<latency>
      mask Display:
      | port_label('input', 1, 'd');
      | port_label('output', 1, 'q');
      | disp(['Z^-', num2str(csp_latency)]);
  pipeline4 : Subsystem  AncestorBlock=casper_library_delays/pipeline  mask(pipeline){csp_latency=1}
      mask prompts: csp_latency "Latency"
      mask help:
      | An explicitly laid-out delay line to avoid mapping to SRL16s
      | for use in pipelining to help achieve timing closure.
      mask init:
      | pipeline_init(gcb,'latency',csp_latency);
      settings: AttributesFormatString=Latency = %<latency>
      mask Display:
      | port_label('input', 1, 'd');
      | port_label('output', 1, 'q');
      | disp(['Z^-', num2str(csp_latency)]);
  pipeline5 : Subsystem  AncestorBlock=casper_library_delays/pipeline  mask(pipeline){csp_latency=1}
      mask prompts: csp_latency "Latency"
      mask help:
      | An explicitly laid-out delay line to avoid mapping to SRL16s
      | for use in pipelining to help achieve timing closure.
      mask init:
      | pipeline_init(gcb,'latency',csp_latency);
      settings: AttributesFormatString=Latency = %<latency>
      mask Display:
      | port_label('input', 1, 'd');
      | port_label('output', 1, 'q');
      | disp(['Z^-', num2str(csp_latency)]);
  pipeline6 : Subsystem  AncestorBlock=casper_library_delays/pipeline  mask(pipeline){csp_latency=1}
      mask prompts: csp_latency "Latency"
      mask help:
      | An explicitly laid-out delay line to avoid mapping to SRL16s
      | for use in pipelining to help achieve timing closure.
      mask init:
      | pipeline_init(gcb,'latency',csp_latency);
      settings: AttributesFormatString=Latency = %<latency>
      mask Display:
      | port_label('input', 1, 'd');
      | port_label('output', 1, 'q');
      | disp(['Z^-', num2str(csp_latency)]);
  pipeline7 : Subsystem  AncestorBlock=casper_library_delays/pipeline  mask(pipeline){csp_latency=1}
      mask prompts: csp_latency "Latency"
      mask help:
      | An explicitly laid-out delay line to avoid mapping to SRL16s
      | for use in pipelining to help achieve timing closure.
      mask init:
      | pipeline_init(gcb,'latency',csp_latency);
      settings: AttributesFormatString=Latency = %<latency>
      mask Display:
      | port_label('input', 1, 'd');
      | port_label('output', 1, 'q');
      | disp(['Z^-', num2str(csp_latency)]);
  pipeline8 : Subsystem  AncestorBlock=casper_library_delays/pipeline  mask(pipeline){csp_latency=2}
      mask prompts: csp_latency "Latency"
      mask help:
      | An explicitly laid-out delay line to avoid mapping to SRL16s
      | for use in pipelining to help achieve timing closure.
      mask init:
      | pipeline_init(gcb,'latency',csp_latency);
      settings: AttributesFormatString=Latency = %<latency>
      mask Display:
      | port_label('input', 1, 'd');
      | port_label('output', 1, 'q');
      | disp(['Z^-', num2str(csp_latency)]);
  pipeline9 : Subsystem  AncestorBlock=casper_library_delays/pipeline  mask(pipeline){csp_latency=1}
      mask prompts: csp_latency "Latency"
      mask help:
      | An explicitly laid-out delay line to avoid mapping to SRL16s
      | for use in pipelining to help achieve timing closure.
      mask init:
      | pipeline_init(gcb,'latency',csp_latency);
      settings: AttributesFormatString=Latency = %<latency>
      mask Display:
      | port_label('input', 1, 'd');
      | port_label('output', 1, 'q');
      | disp(['Z^-', num2str(csp_latency)]);
  posedge1 : Subsystem  AncestorBlock=casper_library_misc/edge_detect  mask(edge_detect){edge=Rising, polarity=Active High, x_in=[0 0.08 0.08 0.16 0.16 0.24 0.24 0.32 0.32 0.4], y_in=[-1 -1  1  1  1  1  1  1  1  1], x_out=[0.6 0.68 0.68 0.76 0.76 0.84 0.84 0.92 0.92 1], y_out=[-1 -1  1  1 -1 -1 -1 -1 -1 -1]}
      mask prompts: edge "Edge Type"; polarity "Output Polarity"; x_in "Input X Positions"; y_in "Input Y Positions"; x_out "Output X Positions"; y_out "Output Y Positions"
      mask help: Output is active for one-cycle after each edge of the specified type (i.e. rising, falling or both).
      mask init:
      | edge_detect_init(gcb,...
      |     'edge',edge,...
      |     'polarity',polarity,...
      |     'x_in',x_in,...
      |     'x_out',x_out,...
      |     'y_in',y_in,...
      |     'y_out',y_out);
      | 
      | x_in_num=str2num(getfield(getfield(get_param(gcb,'UserData'),'parameters'),'x_in'));
      | x_out_num=str2num(getfield(getfield(get_param(gcb,'UserData'),'parameters'),'x_out'));
      | y_in_num=str2num(getfield(getfield(get_param(gcb,'UserData'),'parameters'),'y_in'));
      | y_out_num=str2num(getfield(getfield(get_param(gcb,'UserData'),'parameters'),'y_out'));
      settings: AttributesFormatString=|
      | rising edges
      | active high
      mask Help: Output is active for one-cycle after each edge of the specified type (i.e. rising, falling, or both).  Latency is zero.
      mask TypeOptions edge: Rising | Falling | Both
      mask TypeOptions polarity: Active High | Active Low
      mask Display:
      | plot(x_in_num,0.5+y_in_num*0.2);
      | plot(x_out_num,0.5+y_out_num*0.2);
  rfdc : xps_library/ADCs/rfdc  Tag=xps:rfdc  forceredraw=0  maskopening=1  runinit=1  Tile224_enable=on  t224_enable_mts=off  t224_sample_rate=3932.16  t224_clk_out=245.76  t224_enable_pll=on  t224_ref_clk=245.76  t224_QT_adc0_enable=on  t224_QT_adc0_digital_output=I/Q  t224_QT_adc0_dec_mode=4x  t224_QT_adc0_sample_per_cycle=4  t224_QT_adc0_req_axis_clk=250  t224_QT_adc0_mixer_type=Fine  t224_QT_adc0_mixer_mode=Real -> I/Q  t224_QT_adc0_nco_freq=0  t224_QT_adc0_nco_phase=0  t224_QT_adc0_coarse_freq=0  t224_QT_adc0_nyquist_zone=Zone 1  t224_QT_adc0_cal_mode=Mode 2  t224_QT_adc1_enable=on  t224_QT_adc1_digital_output=I/Q  t224_QT_adc1_dec_mode=4x  t224_QT_adc1_sample_per_cycle=4  t224_QT_adc1_req_axis_clk=250  t224_QT_adc1_mixer_type=Fine  t224_QT_adc1_mixer_mode=Real -> I/Q  t224_QT_adc1_nco_freq=0  t224_QT_adc1_nco_phase=0  t224_QT_adc1_coarse_freq=0  t224_QT_adc1_nyquist_zone=Zone 1  t224_QT_adc1_cal_mode=Mode 2  t224_QT_adc2_enable=on  t224_QT_adc2_digital_output=I/Q  t224_QT_adc2_dec_mode=4x  t224_QT_adc2_sample_per_cycle=4  t224_QT_adc2_req_axis_clk=250  t224_QT_adc2_mixer_type=Fine  t224_QT_adc2_mixer_mode=Real -> I/Q  t224_QT_adc2_nco_freq=0  t224_QT_adc2_nco_phase=0  t224_QT_adc2_coarse_freq=0  t224_QT_adc2_nyquist_zone=Zone 1  t224_QT_adc2_cal_mode=Mode 2  t224_QT_adc3_enable=on  t224_QT_adc3_digital_output=I/Q  t224_QT_adc3_dec_mode=4x  t224_QT_adc3_sample_per_cycle=4  t224_QT_adc3_req_axis_clk=250  t224_QT_adc3_mixer_type=Fine  t224_QT_adc3_mixer_mode=Real -> I/Q  t224_QT_adc3_nco_freq=0  t224_QT_adc3_nco_phase=0  t224_QT_adc3_coarse_freq=0  t224_QT_adc3_nyquist_zone=Zone 1  t224_QT_adc3_cal_mode=Mode 2  t224_DT_adc0_enable=on  t224_DT_adc0_digital_output=Real  t224_DT_adc0_dec_mode=8x  t224_DT_adc0_sample_per_cycle=2  t224_DT_adc0_req_axis_clk=245.76  t224_DT_adc0_mixer_type=Bypassed  t224_DT_adc0_mixer_mode=Real -> Real  t224_DT_adc0_nco_freq=0  t224_DT_adc0_nco_phase=0  t224_DT_adc0_coarse_freq=0  t224_DT_adc0_nyquist_zone=Zone 1  t224_DT_adc0_cal_mode=Mode 2  t224_DT_adc1_enable=on  t224_DT_adc1_digital_output=Real  t224_DT_adc1_dec_mode=8x  t224_DT_adc1_sample_per_cycle=2  t224_DT_adc1_req_axis_clk=245.76  t224_DT_adc1_mixer_type=Bypassed  t224_DT_adc1_mixer_mode=Real -> Real  t224_DT_adc1_nco_freq=0  t224_DT_adc1_nco_phase=0  t224_DT_adc1_coarse_freq=0  t224_DT_adc1_nyquist_zone=Zone 1  t224_DT_adc1_cal_mode=Mode 2  Tile225_enable=off  t225_enable_mts=off  t225_sample_rate=2000  t225_clk_out=125  t225_enable_pll=on  t225_ref_clk=250  t225_QT_adc0_enable=on  t225_QT_adc0_digital_output=Real  t225_QT_adc0_dec_mode=4x  t225_QT_adc0_sample_per_cycle=2  t225_QT_adc0_req_axis_clk=250  t225_QT_adc0_mixer_type=Bypassed  t225_QT_adc0_mixer_mode=Real -> Real  t225_QT_adc0_nco_freq=0  t225_QT_adc0_nco_phase=0  t225_QT_adc0_coarse_freq=0  t225_QT_adc0_nyquist_zone=Zone 1  t225_QT_adc0_cal_mode=Mode 2  t225_QT_adc1_enable=off  t225_QT_adc1_digital_output=Real  t225_QT_adc1_dec_mode=4x  t225_QT_adc1_sample_per_cycle=2  t225_QT_adc1_req_axis_clk=250  t225_QT_adc1_mixer_type=Bypassed  t225_QT_adc1_mixer_mode=Real -> Real  t225_QT_adc1_nco_freq=0  t225_QT_adc1_nco_phase=0  t225_QT_adc1_coarse_freq=0  t225_QT_adc1_nyquist_zone=Zone 1  t225_QT_adc1_cal_mode=Mode 2  t225_QT_adc2_enable=off  t225_QT_adc2_digital_output=Real  t225_QT_adc2_dec_mode=4x  t225_QT_adc2_sample_per_cycle=2  t225_QT_adc2_req_axis_clk=250  t225_QT_adc2_mixer_type=Bypassed  t225_QT_adc2_mixer_mode=Real -> Real  t225_QT_adc2_nco_freq=0  t225_QT_adc2_nco_phase=0  t225_QT_adc2_coarse_freq=0  t225_QT_adc2_nyquist_zone=Zone 1  t225_QT_adc2_cal_mode=Mode 2  t225_QT_adc3_enable=off  t225_QT_adc3_digital_output=Real  t225_QT_adc3_dec_mode=4x  t225_QT_adc3_sample_per_cycle=2  t225_QT_adc3_req_axis_clk=250  t225_QT_adc3_mixer_type=Bypassed  t225_QT_adc3_mixer_mode=Real -> Real  t225_QT_adc3_nco_freq=0  t225_QT_adc3_nco_phase=0  t225_QT_adc3_coarse_freq=0  t225_QT_adc3_nyquist_zone=Zone 1  t225_QT_adc3_cal_mode=Mode 2  t225_DT_adc0_enable=off  t225_DT_adc0_digital_output=Real  t225_DT_adc0_dec_mode=2x  t225_DT_adc0_sample_per_cycle=8  t225_DT_adc0_req_axis_clk=125  t225_DT_adc0_mixer_type=Bypassed  t225_DT_adc0_mixer_mode=Real -> Real  t225_DT_adc0_nco_freq=0  t225_DT_adc0_nco_phase=0  t225_DT_adc0_coarse_freq=0  t225_DT_adc0_nyquist_zone=Zone 1  t225_DT_adc0_cal_mode=Mode 2  t225_DT_adc1_enable=off  t225_DT_adc1_digital_output=Real  t225_DT_adc1_dec_mode=2x  t225_DT_adc1_sample_per_cycle=8  t225_DT_adc1_req_axis_clk=125  t225_DT_adc1_mixer_type=Bypassed  t225_DT_adc1_mixer_mode=Real -> Real  t225_DT_adc1_nco_freq=0  t225_DT_adc1_nco_phase=0  t225_DT_adc1_coarse_freq=0  t225_DT_adc1_nyquist_zone=Zone 1  t225_DT_adc1_cal_mode=Mode 2  Tile226_enable=off  t226_enable_mts=off  t226_sample_rate=2000  t226_clk_out=125  t226_enable_pll=on  t226_ref_clk=250  t226_QT_adc0_enable=on  t226_QT_adc0_digital_output=Real  t226_QT_adc0_dec_mode=4x  t226_QT_adc0_sample_per_cycle=2  t226_QT_adc0_req_axis_clk=250  t226_QT_adc0_mixer_type=Bypassed  t226_QT_adc0_mixer_mode=Real -> Real  t226_QT_adc0_nco_freq=0  t226_QT_adc0_nco_phase=0  t226_QT_adc0_coarse_freq=0  t226_QT_adc0_nyquist_zone=Zone 1  t226_QT_adc0_cal_mode=Mode 2  t226_QT_adc1_enable=off  t226_QT_adc1_digital_output=Real  t226_QT_adc1_dec_mode=4x  t226_QT_adc1_sample_per_cycle=2  t226_QT_adc1_req_axis_clk=250  t226_QT_adc1_mixer_type=Bypassed  t226_QT_adc1_mixer_mode=Real -> Real  t226_QT_adc1_nco_freq=0  t226_QT_adc1_nco_phase=0  t226_QT_adc1_coarse_freq=0  t226_QT_adc1_nyquist_zone=Zone 1  t226_QT_adc1_cal_mode=Mode 2  t226_QT_adc2_enable=off  t226_QT_adc2_digital_output=Real  t226_QT_adc2_dec_mode=4x  t226_QT_adc2_sample_per_cycle=2  t226_QT_adc2_req_axis_clk=250  t226_QT_adc2_mixer_type=Bypassed  t226_QT_adc2_mixer_mode=Real -> Real  t226_QT_adc2_nco_freq=0  t226_QT_adc2_nco_phase=0  t226_QT_adc2_coarse_freq=0  t226_QT_adc2_nyquist_zone=Zone 1  t226_QT_adc2_cal_mode=Mode 2  t226_QT_adc3_enable=off  t226_QT_adc3_digital_output=Real  t226_QT_adc3_dec_mode=4x  t226_QT_adc3_sample_per_cycle=2  t226_QT_adc3_req_axis_clk=250  t226_QT_adc3_mixer_type=Bypassed  t226_QT_adc3_mixer_mode=Real -> Real  t226_QT_adc3_nco_freq=0  t226_QT_adc3_nco_phase=0  t226_QT_adc3_coarse_freq=0  t226_QT_adc3_nyquist_zone=Zone 1  t226_QT_adc3_cal_mode=Mode 2  t226_DT_adc0_enable=off  t226_DT_adc0_digital_output=Real  t226_DT_adc0_dec_mode=2x  t226_DT_adc0_sample_per_cycle=8  t226_DT_adc0_req_axis_clk=125  t226_DT_adc0_mixer_type=Bypassed  t226_DT_adc0_mixer_mode=Real -> Real  t226_DT_adc0_nco_freq=0  t226_DT_adc0_nco_phase=0  t226_DT_adc0_coarse_freq=0  t226_DT_adc0_nyquist_zone=Zone 1  t226_DT_adc0_cal_mode=Mode 2  t226_DT_adc1_enable=off  t226_DT_adc1_digital_output=Real  t226_DT_adc1_dec_mode=2x  t226_DT_adc1_sample_per_cycle=8  t226_DT_adc1_req_axis_clk=125  t226_DT_adc1_mixer_type=Bypassed  t226_DT_adc1_mixer_mode=Real -> Real  t226_DT_adc1_nco_freq=0  t226_DT_adc1_nco_phase=0  t226_DT_adc1_coarse_freq=0  t226_DT_adc1_nyquist_zone=Zone 1  t226_DT_adc1_cal_mode=Mode 2  Tile227_enable=off  t227_enable_mts=off  t227_sample_rate=2000  t227_clk_out=125  t227_enable_pll=on  t227_ref_clk=250  t227_QT_adc0_enable=on  t227_QT_adc0_digital_output=Real  t227_QT_adc0_dec_mode=4x  t227_QT_adc0_sample_per_cycle=2  t227_QT_adc0_req_axis_clk=250  t227_QT_adc0_mixer_type=Bypassed  t227_QT_adc0_mixer_mode=Real -> Real  t227_QT_adc0_nco_freq=0  t227_QT_adc0_nco_phase=0  t227_QT_adc0_coarse_freq=0  t227_QT_adc0_nyquist_zone=Zone 1  t227_QT_adc0_cal_mode=Mode 2  t227_QT_adc1_enable=off  t227_QT_adc1_digital_output=Real  t227_QT_adc1_dec_mode=4x  t227_QT_adc1_sample_per_cycle=2  t227_QT_adc1_req_axis_clk=250  t227_QT_adc1_mixer_type=Bypassed  t227_QT_adc1_mixer_mode=Real -> Real  t227_QT_adc1_nco_freq=0  t227_QT_adc1_nco_phase=0  t227_QT_adc1_coarse_freq=0  t227_QT_adc1_nyquist_zone=Zone 1  t227_QT_adc1_cal_mode=Mode 2  t227_QT_adc2_enable=off  t227_QT_adc2_digital_output=Real  t227_QT_adc2_dec_mode=4x  t227_QT_adc2_sample_per_cycle=2  t227_QT_adc2_req_axis_clk=250  t227_QT_adc2_mixer_type=Bypassed  t227_QT_adc2_mixer_mode=Real -> Real  t227_QT_adc2_nco_freq=0  t227_QT_adc2_nco_phase=0  t227_QT_adc2_coarse_freq=0  t227_QT_adc2_nyquist_zone=Zone 1  t227_QT_adc2_cal_mode=Mode 2  t227_QT_adc3_enable=off  t227_QT_adc3_digital_output=Real  t227_QT_adc3_dec_mode=4x  t227_QT_adc3_sample_per_cycle=2  t227_QT_adc3_req_axis_clk=250  t227_QT_adc3_mixer_type=Bypassed  t227_QT_adc3_mixer_mode=Real -> Real  t227_QT_adc3_nco_freq=0  t227_QT_adc3_nco_phase=0  t227_QT_adc3_coarse_freq=0  t227_QT_adc3_nyquist_zone=Zone 1  t227_QT_adc3_cal_mode=Mode 2  t227_DT_adc0_enable=off  t227_DT_adc0_digital_output=Real  t227_DT_adc0_dec_mode=2x  t227_DT_adc0_sample_per_cycle=8  t227_DT_adc0_req_axis_clk=125  t227_DT_adc0_mixer_type=Bypassed  t227_DT_adc0_mixer_mode=Real -> Real  t227_DT_adc0_nco_freq=0  t227_DT_adc0_nco_phase=0  t227_DT_adc0_coarse_freq=0  t227_DT_adc0_nyquist_zone=Zone 1  t227_DT_adc0_cal_mode=Mode 2  t227_DT_adc1_enable=off  t227_DT_adc1_digital_output=Real  t227_DT_adc1_dec_mode=2x  t227_DT_adc1_sample_per_cycle=8  t227_DT_adc1_req_axis_clk=125  t227_DT_adc1_mixer_type=Bypassed  t227_DT_adc1_mixer_mode=Real -> Real  t227_DT_adc1_nco_freq=0  t227_DT_adc1_nco_phase=0  t227_DT_adc1_coarse_freq=0  t227_DT_adc1_nyquist_zone=Zone 1  t227_DT_adc1_cal_mode=Mode 2  Tile228_enable=off  t228_enable_mts=off  t228_sample_rate=1024  t228_clk_out=64  t228_enable_pll=on  t228_ref_clk=409.6  t228_output_power=20  t228_QT_dac0_enable=on  t228_QT_dac0_analog_output=Real  t228_QT_dac0_inter_mode=4x  t228_QT_dac0_sample_per_cycle=2  t228_QT_dac0_req_axis_clk=250  t228_QT_dac0_datapath_mode=DUC 0 to Fs/2  t228_QT_dac0_mixer_type=Bypassed  t228_QT_dac0_mixer_mode=Real -> Real  t228_QT_dac0_nco_freq=0  t228_QT_dac0_nco_phase=0  t228_QT_dac0_coarse_freq=0  t228_QT_dac0_nyquist_zone=Zone 1  t228_QT_dac0_decode_mode=SNR Optimized  t228_QT_dac1_enable=on  t228_QT_dac1_analog_output=Real  t228_QT_dac1_inter_mode=4x  t228_QT_dac1_sample_per_cycle=2  t228_QT_dac1_req_axis_clk=250  t228_QT_dac1_datapath_mode=DUC 0 to Fs/2  t228_QT_dac1_mixer_type=Bypassed  t228_QT_dac1_mixer_mode=Real -> Real  t228_QT_dac1_nco_freq=0  t228_QT_dac1_nco_phase=0  t228_QT_dac1_coarse_freq=0  t228_QT_dac1_nyquist_zone=Zone 1  t228_QT_dac1_decode_mode=SNR Optimized  t228_QT_dac2_enable=off  t228_QT_dac2_analog_output=Real  t228_QT_dac2_inter_mode=4x  t228_QT_dac2_sample_per_cycle=2  t228_QT_dac2_req_axis_clk=250  t228_QT_dac2_datapath_mode=DUC 0 to Fs/2  t228_QT_dac2_mixer_type=Bypassed  t228_QT_dac2_mixer_mode=Real -> Real  t228_QT_dac2_nco_freq=0  t228_QT_dac2_nco_phase=0  t228_QT_dac2_coarse_freq=0  t228_QT_dac2_nyquist_zone=Zone 1  t228_QT_dac2_decode_mode=SNR Optimized  t228_QT_dac3_enable=off  t228_QT_dac3_analog_output=Real  t228_QT_dac3_inter_mode=4x  t228_QT_dac3_sample_per_cycle=2  t228_QT_dac3_req_axis_clk=250  t228_QT_dac3_datapath_mode=DUC 0 to Fs/2  t228_QT_dac3_mixer_type=Bypassed  t228_QT_dac3_mixer_mode=Real -> Real  t228_QT_dac3_nco_freq=0  t228_QT_dac3_nco_phase=0  t228_QT_dac3_coarse_freq=0  t228_QT_dac3_nyquist_zone=Zone 1  t228_QT_dac3_decode_mode=SNR Optimized  t228_DT_dac0_enable=off  t228_DT_dac0_analog_output=I/Q  t228_DT_dac0_inter_mode=2x  t228_DT_dac0_sample_per_cycle=7  t228_DT_dac0_req_axis_clk=146.286  t228_DT_dac0_mixer_type=Fine  t228_DT_dac0_mixer_mode=I/Q -> I/Q  t228_DT_dac0_nco_freq=0  t228_DT_dac0_nco_phase=0  t228_DT_dac0_coarse_freq=0  t228_DT_dac0_nyquist_zone=Zone 1  t228_DT_dac0_decode_mode=SNR Optimized  t228_DT_dac1_enable=on  t228_DT_dac1_analog_output=I/Q  t228_DT_dac1_inter_mode=2x  t228_DT_dac1_sample_per_cycle=7  t228_DT_dac1_req_axis_clk=146.286  t228_DT_dac1_mixer_type=Off  t228_DT_dac1_mixer_mode=I/Q -> I/Q  t228_DT_dac1_nco_freq=0  t228_DT_dac1_nco_phase=0  t228_DT_dac1_coarse_freq=0  t228_DT_dac1_nyquist_zone=Zone 1  t228_DT_dac1_decode_mode=SNR Optimized  t228_DT_dac2_enable=off  t228_DT_dac2_analog_output=Real  t228_DT_dac2_inter_mode=2x  t228_DT_dac2_sample_per_cycle=7  t228_DT_dac2_req_axis_clk=73.143  t228_DT_dac2_mixer_type=Bypassed  t228_DT_dac2_mixer_mode=Real -> Real  t228_DT_dac2_nco_freq=0  t228_DT_dac2_nco_phase=0  t228_DT_dac2_coarse_freq=0  t228_DT_dac2_nyquist_zone=Zone 1  t228_DT_dac2_decode_mode=SNR Optimized  t228_DT_dac3_enable=off  t228_DT_dac3_analog_output=Real  t228_DT_dac3_inter_mode=2x  t228_DT_dac3_sample_per_cycle=7  t228_DT_dac3_req_axis_clk=73.143  t228_DT_dac3_mixer_type=Bypassed  t228_DT_dac3_mixer_mode=Real -> Real  t228_DT_dac3_nco_freq=0  t228_DT_dac3_nco_phase=0  t228_DT_dac3_coarse_freq=0  t228_DT_dac3_nyquist_zone=Zone 1  t228_DT_dac3_decode_mode=SNR Optimized  Tile229_enable=on  t229_enable_mts=off  t229_sample_rate=3932.16  t229_clk_out=245.76  t229_enable_pll=on  t229_ref_clk=245.76  t229_output_power=20  t229_QT_dac0_enable=on  t229_QT_dac0_analog_output=Real  t229_QT_dac0_inter_mode=4x  t229_QT_dac0_sample_per_cycle=2  t229_QT_dac0_req_axis_clk=250  t229_QT_dac0_datapath_mode=DUC 0 to Fs/2  t229_QT_dac0_mixer_type=Bypassed  t229_QT_dac0_mixer_mode=Real -> Real  t229_QT_dac0_nco_freq=0  t229_QT_dac0_nco_phase=0  t229_QT_dac0_coarse_freq=0  t229_QT_dac0_nyquist_zone=Zone 1  t229_QT_dac0_decode_mode=SNR Optimized  t229_QT_dac1_enable=off  t229_QT_dac1_analog_output=Real  t229_QT_dac1_inter_mode=4x  t229_QT_dac1_sample_per_cycle=2  t229_QT_dac1_req_axis_clk=250  t229_QT_dac1_datapath_mode=DUC 0 to Fs/2  t229_QT_dac1_mixer_type=Bypassed  t229_QT_dac1_mixer_mode=Real -> Real  t229_QT_dac1_nco_freq=0  t229_QT_dac1_nco_phase=0  t229_QT_dac1_coarse_freq=0  t229_QT_dac1_nyquist_zone=Zone 1  t229_QT_dac1_decode_mode=SNR Optimized  t229_QT_dac2_enable=off  t229_QT_dac2_analog_output=Real  t229_QT_dac2_inter_mode=4x  t229_QT_dac2_sample_per_cycle=2  t229_QT_dac2_req_axis_clk=250  t229_QT_dac2_datapath_mode=DUC 0 to Fs/2  t229_QT_dac2_mixer_type=Bypassed  t229_QT_dac2_mixer_mode=Real -> Real  t229_QT_dac2_nco_freq=0  t229_QT_dac2_nco_phase=0  t229_QT_dac2_coarse_freq=0  t229_QT_dac2_nyquist_zone=Zone 1  t229_QT_dac2_decode_mode=SNR Optimized  t229_QT_dac3_enable=off  t229_QT_dac3_analog_output=Real  t229_QT_dac3_inter_mode=4x  t229_QT_dac3_sample_per_cycle=2  t229_QT_dac3_req_axis_clk=250  t229_QT_dac3_datapath_mode=DUC 0 to Fs/2  t229_QT_dac3_mixer_type=Bypassed  t229_QT_dac3_mixer_mode=Real -> Real  t229_QT_dac3_nco_freq=0  t229_QT_dac3_nco_phase=0  t229_QT_dac3_coarse_freq=0  t229_QT_dac3_nyquist_zone=Zone 1  t229_QT_dac3_decode_mode=SNR Optimized  t229_DT_dac0_enable=off  t229_DT_dac0_analog_output=Real  t229_DT_dac0_inter_mode=2x  t229_DT_dac0_sample_per_cycle=4  t229_DT_dac0_req_axis_clk=491.52  t229_DT_dac0_mixer_type=Bypassed  t229_DT_dac0_mixer_mode=Real -> Real  t229_DT_dac0_nco_freq=0  t229_DT_dac0_nco_phase=0  t229_DT_dac0_coarse_freq=0  t229_DT_dac0_nyquist_zone=Zone 1  t229_DT_dac0_decode_mode=SNR Optimized  t229_DT_dac1_enable=off  t229_DT_dac1_analog_output=Real  t229_DT_dac1_inter_mode=2x  t229_DT_dac1_sample_per_cycle=4  t229_DT_dac1_req_axis_clk=491.52  t229_DT_dac1_mixer_type=Bypassed  t229_DT_dac1_mixer_mode=Real -> Real  t229_DT_dac1_nco_freq=0  t229_DT_dac1_nco_phase=0  t229_DT_dac1_coarse_freq=0  t229_DT_dac1_nyquist_zone=Zone 1  t229_DT_dac1_decode_mode=SNR Optimized  t229_DT_dac2_enable=on  t229_DT_dac2_analog_output=Real  t229_DT_dac2_inter_mode=8x  t229_DT_dac2_sample_per_cycle=2  t229_DT_dac2_req_axis_clk=245.76  t229_DT_dac2_mixer_type=Bypassed  t229_DT_dac2_mixer_mode=Real -> Real  t229_DT_dac2_nco_freq=0  t229_DT_dac2_nco_phase=0  t229_DT_dac2_coarse_freq=0  t229_DT_dac2_nyquist_zone=Zone 1  t229_DT_dac2_decode_mode=SNR Optimized  t229_DT_dac3_enable=on  t229_DT_dac3_analog_output=Real  t229_DT_dac3_inter_mode=8x  t229_DT_dac3_sample_per_cycle=2  t229_DT_dac3_req_axis_clk=245.76  t229_DT_dac3_mixer_type=Bypassed  t229_DT_dac3_mixer_mode=Real -> Real  t229_DT_dac3_nco_freq=0  t229_DT_dac3_nco_phase=0  t229_DT_dac3_coarse_freq=0  t229_DT_dac3_nyquist_zone=Zone 1  t229_DT_dac3_decode_mode=SNR Optimized  Tile230_enable=off  t230_enable_mts=off  t230_sample_rate=2000  t230_clk_out=125  t230_enable_pll=on  t230_ref_clk=250  t230_output_power=20  t230_QT_dac0_enable=on  t230_QT_dac0_analog_output=Real  t230_QT_dac0_inter_mode=4x  t230_QT_dac0_sample_per_cycle=2  t230_QT_dac0_req_axis_clk=250  t230_QT_dac0_datapath_mode=DUC 0 to Fs/2  t230_QT_dac0_mixer_type=Bypassed  t230_QT_dac0_mixer_mode=Real -> Real  t230_QT_dac0_nco_freq=0  t230_QT_dac0_nco_phase=0  t230_QT_dac0_coarse_freq=0  t230_QT_dac0_nyquist_zone=Zone 1  t230_QT_dac0_decode_mode=SNR Optimized  t230_QT_dac1_enable=off  t230_QT_dac1_analog_output=Real  t230_QT_dac1_inter_mode=4x  t230_QT_dac1_sample_per_cycle=2  t230_QT_dac1_req_axis_clk=250  t230_QT_dac1_datapath_mode=DUC 0 to Fs/2  t230_QT_dac1_mixer_type=Bypassed  t230_QT_dac1_mixer_mode=Real -> Real  t230_QT_dac1_nco_freq=0  t230_QT_dac1_nco_phase=0  t230_QT_dac1_coarse_freq=0  t230_QT_dac1_nyquist_zone=Zone 1  t230_QT_dac1_decode_mode=SNR Optimized  t230_QT_dac2_enable=off  t230_QT_dac2_analog_output=Real  t230_QT_dac2_inter_mode=4x  t230_QT_dac2_sample_per_cycle=2  t230_QT_dac2_req_axis_clk=250  t230_QT_dac2_datapath_mode=DUC 0 to Fs/2  t230_QT_dac2_mixer_type=Bypassed  t230_QT_dac2_mixer_mode=Real -> Real  t230_QT_dac2_nco_freq=0  t230_QT_dac2_nco_phase=0  t230_QT_dac2_coarse_freq=0  t230_QT_dac2_nyquist_zone=Zone 1  t230_QT_dac2_decode_mode=SNR Optimized  t230_QT_dac3_enable=off  t230_QT_dac3_analog_output=Real  t230_QT_dac3_inter_mode=4x  t230_QT_dac3_sample_per_cycle=2  t230_QT_dac3_req_axis_clk=250  t230_QT_dac3_datapath_mode=DUC 0 to Fs/2  t230_QT_dac3_mixer_type=Bypassed  t230_QT_dac3_mixer_mode=Real -> Real  t230_QT_dac3_nco_freq=0  t230_QT_dac3_nco_phase=0  t230_QT_dac3_coarse_freq=0  t230_QT_dac3_nyquist_zone=Zone 1  t230_QT_dac3_decode_mode=SNR Optimized  Tile231_enable=off  t231_enable_mts=off  t231_sample_rate=2000  t231_clk_out=125  t231_enable_pll=on  t231_ref_clk=250  t231_output_power=20  t231_QT_dac0_enable=on  t231_QT_dac0_analog_output=Real  t231_QT_dac0_inter_mode=4x  t231_QT_dac0_sample_per_cycle=2  t231_QT_dac0_req_axis_clk=250  t231_QT_dac0_datapath_mode=DUC 0 to Fs/2  t231_QT_dac0_mixer_type=Bypassed  t231_QT_dac0_mixer_mode=Real -> Real  t231_QT_dac0_nco_freq=0  t231_QT_dac0_nco_phase=0  t231_QT_dac0_coarse_freq=0  t231_QT_dac0_nyquist_zone=Zone 1  t231_QT_dac0_decode_mode=SNR Optimized  t231_QT_dac1_enable=off  t231_QT_dac1_analog_output=Real  t231_QT_dac1_inter_mode=4x  t231_QT_dac1_sample_per_cycle=2  t231_QT_dac1_req_axis_clk=250  t231_QT_dac1_datapath_mode=DUC 0 to Fs/2  t231_QT_dac1_mixer_type=Bypassed  t231_QT_dac1_mixer_mode=Real -> Real  t231_QT_dac1_nco_freq=0  t231_QT_dac1_nco_phase=0  t231_QT_dac1_coarse_freq=0  t231_QT_dac1_nyquist_zone=Zone 1  t231_QT_dac1_decode_mode=SNR Optimized  t231_QT_dac2_enable=off  t231_QT_dac2_analog_output=Real  t231_QT_dac2_inter_mode=4x  t231_QT_dac2_sample_per_cycle=2  t231_QT_dac2_req_axis_clk=250  t231_QT_dac2_datapath_mode=DUC 0 to Fs/2  t231_QT_dac2_mixer_type=Bypassed  t231_QT_dac2_mixer_mode=Real -> Real  t231_QT_dac2_nco_freq=0  t231_QT_dac2_nco_phase=0  t231_QT_dac2_coarse_freq=0  t231_QT_dac2_nyquist_zone=Zone 1  t231_QT_dac2_decode_mode=SNR Optimized  t231_QT_dac3_enable=off  t231_QT_dac3_analog_output=Real  t231_QT_dac3_inter_mode=4x  t231_QT_dac3_sample_per_cycle=2  t231_QT_dac3_req_axis_clk=250  t231_QT_dac3_datapath_mode=DUC 0 to Fs/2  t231_QT_dac3_mixer_type=Bypassed  t231_QT_dac3_mixer_mode=Real -> Real  t231_QT_dac3_nco_freq=0  t231_QT_dac3_nco_phase=0  t231_QT_dac3_coarse_freq=0  t231_QT_dac3_nyquist_zone=Zone 1  t231_QT_dac3_decode_mode=SNR Optimized  t224_has_adc_clk=off  t224_adc_clk_src=226  t224_clk_dist=None  t225_has_adc_clk=on  t225_adc_clk_src=226  t225_clk_dist=None  t226_has_adc_clk=on  t226_adc_clk_src=226  t226_clk_dist=Input Refclk  t227_has_adc_clk=off  t227_adc_clk_src=226  t227_clk_dist=None  t228_has_dac_clk=off  t228_dac_clk_src=230  t228_clk_dist=None  t229_has_dac_clk=on  t229_dac_clk_src=230  t229_clk_dist=None  t230_has_dac_clk=on  t230_dac_clk_src=230  t230_clk_dist=Input Refclk  t231_has_dac_clk=off  t231_dac_clk_src=230  t231_clk_dist=None  maskdoneopening=0
      settings: SourceProductName=CASPER XPS Blockset
  ri_to_c4 : casper_library_misc/ri_to_c
      settings: SourceProductName=CASPER DSP Blockset
  ri_to_c5 : casper_library_misc/ri_to_c
      settings: SourceProductName=CASPER DSP Blockset
  sync : Subsystem  Tag=xps:sw_reg  AncestorBlock=xps_library/Memory/software_register  mask(swreg){io_dir=From Processor, io_delay=0, init_val=0, sample_period=1, names=reg, bitwidths=1, bin_pts=0, arith_types=2, sim_port=on, show_format=on}
      mask prompts: io_dir "I/O direction"; io_delay "I/O delay"; init_val "Initial Value"; sample_period "Sample period"; names "Bitfield names [msb...lsb]"; bitwidths "Bitfield widths"; bin_pts "Bitfield binary pts"; arith_types "Bitfield types, ufix=0, fix=1, bool=2"; sim_port "Provide sim input/output?"; show_format "Print format string?"
      mask help: A 32-bit software-accessible register. Can be divided into bitfields of varying widths and types using the fields in the block mask.
      mask init:
      | swreg_init(gcb)
      settings: AttributesFormatString=1input:b = 1 bits
      mask TypeOptions io_dir: To Processor | From Processor
      mask Callback io_dir:
      | mask_enables = get_param(gcb, 'MaskEnables');
      | mask_names = get_param(gcb, 'MaskNames');
      | if strcmp(get_param(gcb, 'io_dir'), 'To Processor'),
      |     mask_enables{ismember(mask_names, 'sample_period')} = 'off';
      | else
      |     mask_enables{ismember(mask_names, 'sample_period')} = 'on';
      | end
      | set_param(gcb, 'MaskEnables', mask_enables);
      mask DialogControl ParameterTabVar0 Prompt: Setup
  tge : Subsystem
  wires:
  PFB/1(sync_out) -> chan_reorder/1(sync), fft_sync1/1(sync_in)
  chan_reorder/1(sync_out) -> Counter1/1, Counter4/1, Delay3/1
  DDC/3(i1q1_out) -> c_to_ri1/1, concatenate2/2
  DDC/2(i0q0_out) -> concatenate2/1, c_to_ri7/1
  ri_to_c4/1 -> pipeline7/1(d)
  PFB/2(i0q0) -> concatenate1/1, concatenate7/1
  c_to_ri7/2 -> downsamp/3(q0)
  posedge1/1(out) -> Counter3/1, Counter/1, PFB/1(sync)
  pipeline5/1(q) -> ri_to_c5/2
  ri_to_c5/1 -> pipeline9/1(d)
  c_to_ri1/2 -> downsamp/5(q1)
  pipeline3/1(q) -> ri_to_c5/1
  PFB/3(i1q1) -> concatenate7/2, concatenate1/2
  pipeline4/1(q) -> ri_to_c4/1
  pipeline8/1(q) -> posedge1/1(in)
  pipeline7/1(q) -> PFB/2(i0q0_in)
  pipeline6/1(q) -> ri_to_c4/2
  accum_len/1(in_reg) -> downsamp/7(acc_len_in)
  c_to_ri1/1 -> downsamp/4(i1)
  pipeline9/1(q) -> PFB/3(i1q1_in)
  concatenate7/1 -> chan_reorder/2(din)
  c_to_ri7/1 -> downsamp/2(i0)
  accum_rst/1(in_reg) -> packetize/3(acc_rst_in), downsamp/6(acc_rst_in)
  bus_create/1(bus_out) -> pipeline1/1(d)
  bus_create1/1(bus_out) -> pipeline2/1(d)
  bus_expand/1(msb_out2) -> [adc_i1]
  bus_expand/2(lsb_out1) -> [adc_i0]
  bus_expand1/2(lsb_out1) -> [adc_q0]
  bus_expand1/1(msb_out2) -> [adc_q1]
  [adc_i1] -> pipeline3/1(d)
  [adc_i0] -> pipeline4/1(d)
  [adc_q1] -> pipeline5/1(d)
  [adc_q0] -> pipeline6/1(d)
  sync/1(in_reg) -> edge_detect/1
  [sync] -> pipeline8/1(d)
  edge_detect/1 -> [sync]
  fft_shift/1(in_reg) -> [fft_shift]
  [fft_shift] -> PFB/4(fft_shift_in)
  concatenate1/1 -> bus_convert/1(din)
  bus_convert/1(dout) -> Delay1/1
  Constant/1 -> pfb_snapshot/2(we)
  [dac_i1] -> bus_create/1(in1)
  [dac_i0] -> bus_create/2(in2)
  [dac_q0] -> bus_create1/2(in2)
  [dac_q1] -> bus_create1/1(in1)
  Counter/1 -> dac_wave_i/1(addr)
  Constant1/1 -> dac_wave_i/2(data_in)
  Constant2/1 -> dac_wave_i/3(we)
  dac_wave_i/1(data_out) -> pipeline13/1(d)
  dds_wave_i/1(data_out) -> pipeline14/1(d)
  Constant4/1 -> dds_wave_i/3(we)
  Constant3/1 -> dds_wave_i/2(data_in)
  Counter1/1 -> dds_wave_i/1(addr)
  [dds_i0] -> DDC/4(dds_i0)
  [dds_i1] -> DDC/5(dds_i1)
  PFB/4("fft_of ") -> Counter2/1
  Counter2/1 -> fft_of_cnt/1(out_reg)
  bus_convert1/1(dout) -> Delay4/1
  Constant5/1 -> ddc_snapshot/2(we)
  concatenate2/1 -> bus_convert1/1(din)
  DDC/1("sync_out ") -> downsamp/1(sync_in), fft_sync2/1(sync_in)
  rfdc/1 -> pipeline10/1(d)
  Constant6/1 -> acc_snapshot0/2(we)
  bus_create2/1(bus_out) -> acc_snapshot0/1(din)
  downsamp/1(i0_out) -> [vacc_i0]
  downsamp/2(q0_out) -> [vacc_q0]
  downsamp/3(i1_out) -> [vacc_i1]
  downsamp/4(q1_out) -> [vacc_q1]
  downsamp/5(new_acc) -> [new_acc]
  [new_acc] -> acc_snapshot0/3(trig)
  [new_acc] -> acc_snapshot1/3(trig)
  bus_create3/1(bus_out) -> acc_snapshot1/1(din)
  Constant7/1 -> acc_snapshot1/2(we)
  [vacc_i1] -> bus_create3/1(in1)
  [vacc_q1] -> bus_create3/2(in2)
  [vacc_q0] -> bus_create2/2(in2)
  [vacc_i0] -> bus_create2/1(in1)
  acc_snapshot0/1(arm_out) -> acc_snapshot1/4(arm)
  pipeline1/1(q) -> Mux/3, rfdc/3
  pipeline2/1(q) -> Mux1/3, rfdc/4
  bus_create4/1(bus_out) -> pipeline12/1(d)
  Constant8/1 -> adc_snapshot/2(we)
  Constant9/1 -> adc_snapshot/3(trig)
  [adc_i0] -> bus_create4/1(in1)
  [adc_q0] -> bus_create4/2(in2)
  [adc_i1] -> bus_create4/3(in3)
  [adc_q1] -> bus_create4/4(in4)
  pipeline12/1(q) -> adc_snapshot/1(din)
  pipeline10/1(q) -> Mux/2
  Mux/1 -> bus_expand/1(bus_in)
  pipeline11/1(q) -> Mux1/2
  Mux1/1 -> bus_expand1/1(bus_in)
  adc_dac_loopback/1(in_reg) -> Mux1/1, Mux/1
  pipeline13/1(q) -> bus_expand2/1(bus_in)
  pipeline14/1(q) -> bus_expand3/1(bus_in)
  pipeline15/1(q) -> bus_expand4/1(bus_in)
  dac_wave_q/1(data_out) -> pipeline15/1(d)
  Constant11/1 -> dac_wave_q/3(we)
  Constant10/1 -> dac_wave_q/2(data_in)
  Counter3/1 -> dac_wave_q/1(addr)
  bus_expand2/1(msb_out2) -> Reinterpret/1, [dac_i0]
  bus_expand2/2(lsb_out1) -> Reinterpret1/1, [dac_i1]
  bus_expand4/1(msb_out2) -> [dac_q0]
  bus_expand4/2(lsb_out1) -> [dac_q1]
  pipeline16/1(q) -> bus_expand5/1(bus_in)
  Counter4/1 -> dds_wave_q/1(addr)
  Constant12/1 -> dds_wave_q/2(data_in)
  Constant13/1 -> dds_wave_q/3(we)
  dds_wave_q/1(data_out) -> pipeline16/1(d)
  bus_expand3/1(msb_out2) -> [dds_i0]
  bus_expand3/2(lsb_out1) -> [dds_i1]
  bus_expand5/1(msb_out2) -> [dds_q0]
  bus_expand5/2(lsb_out1) -> [dds_q1]
  rfdc/2 -> pipeline11/1(d)
  Reinterpret/1 -> dac_readback_msb/1(out_reg)
  Reinterpret1/1 -> dac_readback_lsb/1(out_reg)
  Delay2/1 -> DDC/2(i0q0)
  Delay3/1 -> DDC/1("sync_in ")
  Delay5/1 -> DDC/3(i1q1)
  [dds_q0] -> DDC/6(dds_q0)
  [dds_q1] -> DDC/7(dds_q1)
  chan_reorder/2(dout) -> bus_expand6/1(bus_in)
  bus_expand6/1(msb_out2) -> Delay2/1
  bus_expand6/2(lsb_out1) -> Delay5/1
  [vacc_i0] -> bus_create5/1(in1)
  [vacc_q0] -> bus_create5/2(in2)
  [new_acc] -> Delay9/1, acc_chan0_snapshot/3(trig)
  bus_create5/1(bus_out) -> acc_chan0_snapshot/1(din)
  Delay9/1 -> acc_chan0_snapshot/2(we)
  fft_sync1/1(data_ready) -> pfb_snapshot/3(trig)
  fft_sync2/1(data_ready) -> ddc_snapshot/3(trig)
  Delay1/1 -> pfb_snapshot/1(din)
  Delay4/1 -> ddc_snapshot/1(din)
  packetize/2(vld) -> tge/2(vld)
  packetize/1(dout) -> tge/1(data)
  packetize/3(eof) -> tge/3(eof)
  bus_create6/1(bus_out) -> packetize/2(din)
  [vacc_i0] -> bus_create6/1(in1)
  [vacc_q0] -> bus_create6/2(in2)
  [vacc_i1] -> bus_create6/3(in3)
  [vacc_q1] -> bus_create6/4(in4)
  [new_acc] -> packetize/1(new_acc)
